simulink model "twozonevav"  (R2020a)
settings: Solver=FixedStepAuto  StartTime=0.0  StopTime=Inf  FixedStep=0.001  RelTol=1e-3
PostLoadFcn:
  | if any(exist('dsrtsu_mdlpostloadfcn', 'file') ~= 0), dsrtsu_mdlpostloadfcn('Execute', bdroot); end
InitFcn:
  | , if any(exist('rtifpga_mdlclblib', 'file') ~= 0), rtifpga_mdlclblib('Init', bdroot); end,
  | , if any(exist('dsmpb_private', 'file') ~= 0), dsmpb_private('dsmpb_mdlclblib', 'Init', bdroot); end,
libraries: dsmpblib x8
(part 2 of 3)

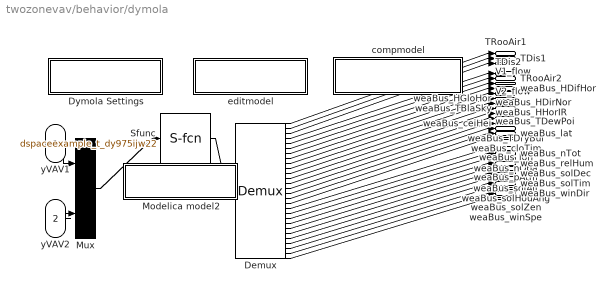
== system twozonevav/behavior/dymola ==
  yVAV1 : Inport
  yVAV2 : Inport  Port=2
  Demux : Demux  Outputs=[1;1;1;1;1;1;1;1;1;1;1;1;1;1;1;1;1;1;1;1;1;1;1;1;1;1;1;1]
  Dymola Settings : Subsystem  mask{ModelName=dSpaceExample.TwoZoneVAV, MoFileName=D:/github/dspace-modelica-example/dSpaceExample/TwoZoneVAV.mo, dSpace=, BusConnector=[], ResultFile=[], ResultFileOnline=[], ResultDt=[], Libs=:, bigobj=[], ImportFolder=[], guimode=[], ModelName2=[], forRuntime=[], MEXLoad=[], omitDescription=[], ResultName=dspaceexample_t_dy975ijw22}
      mask prompts: ModelName "Name of Dymola model"; MoFileName "File Name (including .mo)"; ResultFile "Create Result"; ResultFileOnline "Load result"; ResultDt "Result min dt"; Libs "Used Libraries"; bigobj "Compiler flag /bigobj"; ImportFolder "Import folder"; guimode "GUI mode flag"; ModelName2 "Model name for import mode"; forRuntime "Runtime export"; MEXLoad "Compiled S-function"; omitDescription "Omit description strings"; ResultName "Name of result file"
      mask Display: disp('Dymola Settings');
  Modelica model2 : Subsystem
      mask Display: disp('Change parameters');
  Mux : Mux  Inputs=[1;1]
  Sfunc : S-Function  Tag=975ijw22  FunctionName=dspaceexample_t_dy975ijw22  Parameters=[VRoo;zon1_S_;zon1_E_;zon1_W_;zon1_N_;zon1_matExtWal_absIR_a;zon1_matExtWal_absIR_b;zon1_matExtWal_absSol_a;zon1_matExtWal_absSol_b;zon1_matExtWal_roughness_10;zon1_matFlo_absIR_a;zon1_matFlo_absIR_b;zon1_matFlo_absSol_a;zon1_matFlo_absSol_b;zon1_matFlo_roughness_a;zon1_roof_absIR_a;zon1_roof_absIR_b;zon1_roof_absSol_a;zon1_roof_absSol_b;zon1_roof_roughness_a;zon1_window600_glass_1__x;zon1_window600_glass_1__k;zon1_window600_glass_1__t23;zon1_window600_glass_1__r24;zon1_window600_glass_1__r25;zon1_window600_glass_1__t26;zon1_window600_glass_1__a27;zon1_window600_glass_1__a28;zon1_window600_glass_2__x;zon1_window600_glass_2__k;zon1_window600_glass_2__t31;zon1_window600_glass_2__r32;zon1_window600_glass_2__r33;zon1_window600_glass_2__t34;zon1_window600_glass_2__a35;zon1_window600_glass_2__a36;zon1_window600_gas_1__x;zon1_window600_gas_1__a_k;zon1_window600_gas_1__b_k;zon1_window600_gas_1__a_m40;zon1_window600_gas_1__b_m41;zon1_window600_gas_1__a_c;zon1_window600_gas_1__b_c;zon1_window600_gas_1__MM;zon1_window600_gas_1__P0;zon1_window600_shade_tauS46;zon1_window600_shade_tauS47;zon1_window600_shade_rhoS48;zon1_window600_shade_rhoS49;zon1_window600_shade_absI50;zon1_window600_shade_absI51;zon1_window600_shade_tauI52;zon1_window600_shade_tauI53;zon1_window600_UFra;zon1_window600_absIRFra;zon1_window600_absSolFra;zon1_soi_A;zon1_soi_T_a_start;zon1_soi_T_b_start;zon1_roo_datConExt_1__bou60;zon1_roo_datConExt_1__A;zon1_roo_datConExt_2__bou62;zon1_roo_datConExt_2__A;zon1_roo_datConExt_3__bou64;zon1_roo_datConExt_3__A;zon1_roo_datConExt_4__bou66;zon1_roo_datConExt_4__A;zon1_roo_datConExtWin_1__68;zon1_roo_datConExtWin_1__69;zon1_roo_datConExtWin_1__70;zon1_roo_datConExtWin_1__71;zon1_roo_datConExtWin_1__72;zon1_roo_datConExtWin_1__73;zon1_roo_datConExtWin_1__74;zon1_roo_datConExtWin_1__75;zon1_roo_datConExtWin_1__76;zon1_roo_datConExtWin_1__77;zon1_roo_datConPar_1__azi;zon1_roo_datConPar_1__bou79;zon1_roo_datConPar_1__A;zon1_roo_datConBou_1__azi;zon1_roo_datConBou_1__bou82;zon1_roo_datConBou_1__A;zon1_roo_surBou_1__A;zon1_roo_surBou_1__absIR;zon1_roo_surBou_1__absSol;zon1_roo_surBou_1__bounda87;zon1_roo_dummyCon_absIR_a;zon1_roo_dummyCon_absIR_b;zon1_roo_dummyCon_absSol_90;zon1_roo_dummyCon_absSol_91;zon1_roo_dummyCon_roughne92;zon1_roo_dummyGlaSys_glas93;zon1_roo_dummyGlaSys_glas94;zon1_roo_dummyGlaSys_glas95;zon1_roo_dummyGlaSys_glas96;zon1_roo_dummyGlaSys_glas97;zon1_roo_dummyGlaSys_glas98;zon1_roo_dummyGlaSys_glas99;zon1_roo_dummyGlaSys_glas100;zon1_roo_dummyGlaSys_gas_101;zon1_roo_dummyGlaSys_gas_102;zon1_roo_dummyGlaSys_gas_103;zon1_roo_dummyGlaSys_gas_104;zon1_roo_dummyGlaSys_gas_105;zon1_roo_dummyGlaSys_gas_106;zon1_roo_dummyGlaSys_gas_107;zon1_roo_dummyGlaSys_gas_108;zon1_roo_dummyGlaSys_gas_109;zon1_roo_dummyGlaSys_shad110;zon1_roo_dummyGlaSys_shad111;zon1_roo_dummyGlaSys_shad112;zon1_roo_dummyGlaSys_shad113;zon1_roo_dummyGlaSys_shad114;zon1_roo_dummyGlaSys_shad115;zon1_roo_dummyGlaSys_shad116;zon1_roo_dummyGlaSys_shad117;zon1_roo_dummyGlaSys_UFra;zon1_roo_dummyGlaSys_absI119;zon1_roo_dummyGlaSys_absS120;zon1_roo_AFlo;zon1_roo_hRoo;zon1_roo_conExtWin_1__gla123;zon1_roo_conExtWin_1__win124;zon1_roo_conExtWin_1__win125;zon1_roo_conExtWin_1__win126;zon1_roo_conExtWin_1__win127;zon1_roo_hIntFixed;zon1_roo_hExtFixed;zon1_roo_bouConExt_HDifTi130;zon1_roo_bouConExt_HDifTi131;zon1_roo_bouConExt_HDifTi132;zon1_roo_bouConExt_HDifTi133;zon1_roo_bouConExt_HDifTi134;zon1_roo_bouConExt_HDifTi135;zon1_roo_bouConExt_HDifTi136;zon1_roo_bouConExt_HDifTi137;zon1_roo_bouConExt_HDifTi138;zon1_roo_bouConExt_HDifTi139;zon1_roo_bouConExt_HDifTi140;zon1_roo_bouConExt_HDifTi141;zon1_roo_bouConExtWin_con142;zon1_roo_bouConExtWin_con143;zon1_roo_bouConExtWin_HDi144;zon1_roo_bouConExtWin_HDi145;zon1_roo_bouConExtWin_HDi146;zon1_roo_bouConExtWin_con147;zon1_roo_air_datConExtWin148;zon1_roo_air_datConExtWin149;zon1_roo_air_dummyCon_abs150;zon1_roo_air_dummyCon_abs151;zon1_roo_air_dummyCon_abs152;zon1_roo_air_dummyCon_abs153;zon1_roo_air_dummyCon_rou154;zon1_roo_air_dummyGlaSys_155;zon1_roo_air_dummyGlaSys_156;zon1_roo_air_dummyGlaSys_157;zon1_roo_air_dummyGlaSys_158;zon1_roo_air_dummyGlaSys_159;zon1_roo_air_dummyGlaSys_160;zon1_roo_air_dummyGlaSys_161;zon1_roo_air_dummyGlaSys_162;zon1_roo_air_dummyGlaSys_163;zon1_roo_air_dummyGlaSys_164;zon1_roo_air_dummyGlaSys_165;zon1_roo_air_dummyGlaSys_166;zon1_roo_air_dummyGlaSys_167;zon1_roo_air_dummyGlaSys_168;zon1_roo_air_dummyGlaSys_169;zon1_roo_air_dummyGlaSys_170;zon1_roo_air_dummyGlaSys_171;zon1_roo_air_dummyGlaSys_172;zon1_roo_air_dummyGlaSys_173;zon1_roo_air_dummyGlaSys_174;zon1_roo_air_dummyGlaSys_175;zon1_roo_air_dummyGlaSys_176;zon1_roo_air_dummyGlaSys_177;zon1_roo_air_dummyGlaSys_178;zon1_roo_air_dummyGlaSys_179;zon1_roo_air_dummyGlaSys_180;zon1_roo_air_dummyGlaSys_181;zon1_roo_air_dummyGlaSys_182;zon1_roo_solRadExc_datCon183;zon1_roo_solRadExc_datCon184;zon1_roo_solRadExc_dummyC185;zon1_roo_solRadExc_dummyC186;zon1_roo_solRadExc_dummyC187;zon1_roo_solRadExc_dummyC188;zon1_roo_solRadExc_dummyC189;zon1_roo_solRadExc_dummyG190;zon1_roo_solRadExc_dummyG191;zon1_roo_solRadExc_dummyG192;zon1_roo_solRadExc_dummyG193;zon1_roo_solRadExc_dummyG194;zon1_roo_solRadExc_dummyG195;zon1_roo_solRadExc_dummyG196;zon1_roo_solRadExc_dummyG197;zon1_roo_solRadExc_dummyG198;zon1_roo_solRadExc_dummyG199;zon1_roo_solRadExc_dummyG200;zon1_roo_solRadExc_dummyG201;zon1_roo_solRadExc_dummyG202;zon1_roo_solRadExc_dummyG203;zon1_roo_solRadExc_dummyG204;zon1_roo_solRadExc_dummyG205;zon1_roo_solRadExc_dummyG206;zon1_roo_solRadExc_dummyG207;zon1_roo_solRadExc_dummyG208;zon1_roo_solRadExc_dummyG209;zon1_roo_solRadExc_dummyG210;zon1_roo_solRadExc_dummyG211;zon1_roo_solRadExc_dummyG212;zon1_roo_solRadExc_dummyG213;zon1_roo_solRadExc_dummyG214;zon1_roo_solRadExc_dummyG215;zon1_roo_solRadExc_dummyG216;zon1_roo_solRadExc_dummyG217;zon1_roo_irRadGai_datConE218;zon1_roo_irRadGai_datConE219;zon1_roo_irRadGai_dummyCo220;zon1_roo_irRadGai_dummyCo221;zon1_roo_irRadGai_dummyCo222;zon1_roo_irRadGai_dummyCo223;zon1_roo_irRadGai_dummyCo224;zon1_roo_irRadGai_dummyGl225;zon1_roo_irRadGai_dummyGl226;zon1_roo_irRadGai_dummyGl227;zon1_roo_irRadGai_dummyGl228;zon1_roo_irRadGai_dummyGl229;zon1_roo_irRadGai_dummyGl230;zon1_roo_irRadGai_dummyGl231;zon1_roo_irRadGai_dummyGl232;zon1_roo_irRadGai_dummyGl233;zon1_roo_irRadGai_dummyGl234;zon1_roo_irRadGai_dummyGl235;zon1_roo_irRadGai_dummyGl236;zon1_roo_irRadGai_dummyGl237;zon1_roo_irRadGai_dummyGl238;zon1_roo_irRadGai_dummyGl239;zon1_roo_irRadGai_dummyGl240;zon1_roo_irRadGai_dummyGl241;zon1_roo_irRadGai_dummyGl242;zon1_roo_irRadGai_dummyGl243;zon1_roo_irRadGai_dummyGl244;zon1_roo_irRadGai_dummyGl245;zon1_roo_irRadGai_dummyGl246;zon1_roo_irRadGai_dummyGl247;zon1_roo_irRadGai_dummyGl248;zon1_roo_irRadGai_dummyGl249;zon1_roo_irRadGai_dummyGl250;zon1_roo_irRadGai_dummyGl251;zon1_roo_irRadGai_dummyGl252;zon1_roo_irRadExc_datConE253;zon1_roo_irRadExc_datConE254;zon1_roo_irRadExc_dummyCo255;zon1_roo_irRadExc_dummyCo256;zon1_roo_irRadExc_dummyCo257;zon1_roo_irRadExc_dummyCo258;zon1_roo_irRadExc_dummyCo259;zon1_roo_irRadExc_dummyGl260;zon1_roo_irRadExc_dummyGl261;zon1_roo_irRadExc_dummyGl262;zon1_roo_irRadExc_dummyGl263;zon1_roo_irRadExc_dummyGl264;zon1_roo_irRadExc_dummyGl265;zon1_roo_irRadExc_dummyGl266;zon1_roo_irRadExc_dummyGl267;zon1_roo_irRadExc_dummyGl268;zon1_roo_irRadExc_dummyGl269;zon1_roo_irRadExc_dummyGl270;zon1_roo_irRadExc_dummyGl271;zon1_roo_irRadExc_dummyGl272;zon1_roo_irRadExc_dummyGl273;zon1_roo_irRadExc_dummyGl274;zon1_roo_irRadExc_dummyGl275;zon1_roo_irRadExc_dummyGl276;zon1_roo_irRadExc_dummyGl277;zon1_roo_irRadExc_dummyGl278;zon1_roo_irRadExc_dummyGl279;zon1_roo_irRadExc_dummyGl280;zon1_roo_irRadExc_dummyGl281;zon1_roo_irRadExc_dummyGl282;zon1_roo_irRadExc_dummyGl283;zon1_roo_irRadExc_dummyGl284;zon1_roo_irRadExc_dummyGl285;zon1_roo_irRadExc_dummyGl286;zon1_roo_irRadExc_dummyGl287;zon1_roo_irRadExc_T0;zon1_roo_radTem_datConExt289;zon1_roo_radTem_datConExt290;zon1_roo_radTem_dummyCon_291;zon1_roo_radTem_dummyCon_292;zon1_roo_radTem_dummyCon_293;zon1_roo_radTem_dummyCon_294;zon1_roo_radTem_dummyCon_295;zon1_roo_radTem_dummyGlaS296;zon1_roo_radTem_dummyGlaS297;zon1_roo_radTem_dummyGlaS298;zon1_roo_radTem_dummyGlaS299;zon1_roo_radTem_dummyGlaS300;zon1_roo_radTem_dummyGlaS301;zon1_roo_radTem_dummyGlaS302;zon1_roo_radTem_dummyGlaS303;zon1_roo_radTem_dummyGlaS304;zon1_roo_radTem_dummyGlaS305;zon1_roo_radTem_dummyGlaS306;zon1_roo_radTem_dummyGlaS307;zon1_roo_radTem_dummyGlaS308;zon1_roo_radTem_dummyGlaS309;zon1_roo_radTem_dummyGlaS310;zon1_roo_radTem_dummyGlaS311;zon1_roo_radTem_dummyGlaS312;zon1_roo_radTem_dummyGlaS313;zon1_roo_radTem_dummyGlaS314;zon1_roo_radTem_dummyGlaS315;zon1_roo_radTem_dummyGlaS316;zon1_roo_radTem_dummyGlaS317;zon1_roo_radTem_dummyGlaS318;zon1_roo_radTem_dummyGlaS319;zon1_roo_radTem_dummyGlaS320;zon1_roo_radTem_dummyGlaS321;zon1_roo_radTem_dummyGlaS322;zon1_roo_radTem_dummyGlaS323;zon1_roo_add_k1;zon1_roo_add_k2;zon1_roo_sumJFroWin_1__k;zon1_roo_p_start;zon1_roo_T_start;zon1_roo_X_start;zon1_qConGai_flow_k;zon1_qRadGai_flow_k;zon1_qLatGai_flow_k;zon1_TSoi_1__T;zon1_sinInf_m_flow;zon1_sinInf_x_pTphi_p;zon1_InfiltrationRate_k;zon1_souInf_m_flow;zon1_souInf_x_pTphi_p;zon1_intLoad_table;zon1_intLoad_verboseRead;zon1_intLoad_columns;zon1_intLoad_offset;zon1_intLoad_startTime;zon1_intLoad_timeEvents;coiSou_X;coiSou_T;res_sta_default_p;res_sta_default_T;res_sta_default_X;weaDat_lon;weaDat_lat;weaDat_wea_table;weaDat_wea_verboseRead;weaDat_wea_offset;weaDat_wea_startTime;weaDat_wea_timeEvents;sin_X;sin_p;sin_T;vav1_vav_sta_default_p;vav1_vav_sta_default_T;vav1_vav_sta_default_X;vav1_vav_riseTime;vav1_vav_y_start;vav1_vav_filter_gain;vav1_vav_filter_A_ripple;vav1_vav_filter_f_min;vav1_vav_filter_normalize368;vav1_vav_filter_x_start;vav1_vav_filter_u_nominal;vav1_vav_use_deltaM;vav1_vav_deltaM;vav1_vav_roundDuct;vav1_vav_ReC;vav1_vav_a;vav1_vav_b;vav1_vav_yL;vav1_vav_yU;vav1_vav_k1;vav1_vav_l;vav1_vav_l2;vav1_vav_deltax;vav1_vav_y_min;vav1_terHea_bal1_preDro_s384;vav1_terHea_bal1_preDro_s385;vav1_terHea_bal1_preDro_s386;vav1_terHea_bal2_preDro_s387;vav1_terHea_bal2_preDro_s388;vav1_terHea_delta;vav1_terHea_T_a1_nominal;vav1_terHea_T_a2_nominal;vav1_terHea_r_nominal;vav1_terHea_hA_n_w;vav1_terHea_hA_n_a;vav1_terHea_hA_T0_w;vav1_terHea_hA_T0_a;vav1_sinTer_X;vav1_sinTer_p;vav1_sinTer_T;vav1_souTer_X;vav1_souTer_m_flow;vav1_souTer_T;VSup1_T_start;VSup1_p_start;VSup1_X_start;TDisVAV1_T_start;TDisVAV1_TAmb;TDisVAV1_tauHeaTra;zer_k;vav2_vav_sta_default_p;vav2_vav_sta_default_T;vav2_vav_sta_default_X;vav2_vav_riseTime;vav2_vav_y_start;vav2_vav_filter_gain;vav2_vav_filter_A_ripple;vav2_vav_filter_f_min;vav2_vav_filter_normalize418;vav2_vav_filter_x_start;vav2_vav_filter_u_nominal;vav2_vav_use_deltaM;vav2_vav_deltaM;vav2_vav_roundDuct;vav2_vav_ReC;vav2_vav_a;vav2_vav_b;vav2_vav_yL;vav2_vav_yU;vav2_vav_k1;vav2_vav_l;vav2_vav_l2;vav2_vav_deltax;vav2_vav_y_min;vav2_terHea_bal1_preDro_s434;vav2_terHea_bal1_preDro_s435;vav2_terHea_bal1_preDro_s436;vav2_terHea_bal2_preDro_s437;vav2_terHea_bal2_preDro_s438;vav2_terHea_delta;vav2_terHea_T_a1_nominal;vav2_terHea_T_a2_nominal;vav2_terHea_r_nominal;vav2_terHea_hA_n_w;vav2_terHea_hA_n_a;vav2_terHea_hA_T0_w;vav2_terHea_hA_T0_a;vav2_sinTer_X;vav2_sinTer_p;vav2_sinTer_T;vav2_souTer_X;vav2_souTer_m_flow;vav2_souTer_T;TDisVAV2_T_start;TDisVAV2_TAmb;TDisVAV2_tauHeaTra;VSup2_T_start;VSup2_p_start;VSup2_X_start;zon2_S_;zon2_E_;zon2_W_;zon2_N_;zon2_matExtWal_absIR_a;zon2_matExtWal_absIR_b;zon2_matExtWal_absSol_a;zon2_matExtWal_absSol_b;zon2_matExtWal_roughness_467;zon2_matFlo_absIR_a;zon2_matFlo_absIR_b;zon2_matFlo_absSol_a;zon2_matFlo_absSol_b;zon2_matFlo_roughness_a;zon2_roof_absIR_a;zon2_roof_absIR_b;zon2_roof_absSol_a;zon2_roof_absSol_b;zon2_roof_roughness_a;zon2_window600_glass_1__x;zon2_window600_glass_1__k;zon2_window600_glass_1__t480;zon2_window600_glass_1__r481;zon2_window600_glass_1__r482;zon2_window600_glass_1__t483;zon2_window600_glass_1__a484;zon2_window600_glass_1__a485;zon2_window600_glass_2__x;zon2_window600_glass_2__k;zon2_window600_glass_2__t488;zon2_window600_glass_2__r489;zon2_window600_glass_2__r490;zon2_window600_glass_2__t491;zon2_window600_glass_2__a492;zon2_window600_glass_2__a493;zon2_window600_gas_1__x;zon2_window600_gas_1__a_k;zon2_window600_gas_1__b_k;zon2_window600_gas_1__a_m497;zon2_window600_gas_1__b_m498;zon2_window600_gas_1__a_c;zon2_window600_gas_1__b_c;zon2_window600_gas_1__MM;zon2_window600_gas_1__P0;zon2_window600_shade_tauS503;zon2_window600_shade_tauS504;zon2_window600_shade_rhoS505;zon2_window600_shade_rhoS506;zon2_window600_shade_absI507;zon2_window600_shade_absI508;zon2_window600_shade_tauI509;zon2_window600_shade_tauI510;zon2_window600_UFra;zon2_window600_absIRFra;zon2_window600_absSolFra;zon2_soi_A;zon2_soi_T_a_start;zon2_soi_T_b_start;zon2_roo_datConExt_1__bou517;zon2_roo_datConExt_1__A;zon2_roo_datConExt_2__bou519;zon2_roo_datConExt_2__A;zon2_roo_datConExt_3__bou521;zon2_roo_datConExt_3__A;zon2_roo_datConExt_4__bou523;zon2_roo_datConExt_4__A;zon2_roo_datConExtWin_1__525;zon2_roo_datConExtWin_1__526;zon2_roo_datConExtWin_1__527;zon2_roo_datConExtWin_1__528;zon2_roo_datConExtWin_1__529;zon2_roo_datConExtWin_1__530;zon2_roo_datConExtWin_1__531;zon2_roo_datConExtWin_1__532;zon2_roo_datConExtWin_1__533;zon2_roo_datConExtWin_1__534;zon2_roo_datConPar_1__azi;zon2_roo_datConPar_1__bou536;zon2_roo_datConPar_1__A;zon2_roo_datConBou_1__azi;zon2_roo_datConBou_1__bou539;zon2_roo_datConBou_1__A;zon2_roo_surBou_1__A;zon2_roo_surBou_1__absIR;zon2_roo_surBou_1__absSol;zon2_roo_surBou_1__bounda544;zon2_roo_dummyCon_absIR_a;zon2_roo_dummyCon_absIR_b;zon2_roo_dummyCon_absSol_547;zon2_roo_dummyCon_absSol_548;zon2_roo_dummyCon_roughne549;zon2_roo_dummyGlaSys_glas550;zon2_roo_dummyGlaSys_glas551;zon2_roo_dummyGlaSys_glas552;zon2_roo_dummyGlaSys_glas553;zon2_roo_dummyGlaSys_glas554;zon2_roo_dummyGlaSys_glas555;zon2_roo_dummyGlaSys_glas556;zon2_roo_dummyGlaSys_glas557;zon2_roo_dummyGlaSys_gas_558;zon2_roo_dummyGlaSys_gas_559;zon2_roo_dummyGlaSys_gas_560;zon2_roo_dummyGlaSys_gas_561;zon2_roo_dummyGlaSys_gas_562;zon2_roo_dummyGlaSys_gas_563;zon2_roo_dummyGlaSys_gas_564;zon2_roo_dummyGlaSys_gas_565;zon2_roo_dummyGlaSys_gas_566;zon2_roo_dummyGlaSys_shad567;zon2_roo_dummyGlaSys_shad568;zon2_roo_dummyGlaSys_shad569;zon2_roo_dummyGlaSys_shad570;zon2_roo_dummyGlaSys_shad571;zon2_roo_dummyGlaSys_shad572;zon2_roo_dummyGlaSys_shad573;zon2_roo_dummyGlaSys_shad574;zon2_roo_dummyGlaSys_UFra;zon2_roo_dummyGlaSys_absI576;zon2_roo_dummyGlaSys_absS577;zon2_roo_AFlo;zon2_roo_hRoo;zon2_roo_conExtWin_1__gla580;zon2_roo_conExtWin_1__win581;zon2_roo_conExtWin_1__win582;zon2_roo_conExtWin_1__win583;zon2_roo_conExtWin_1__win584;zon2_roo_hIntFixed;zon2_roo_hExtFixed;zon2_roo_bouConExt_HDifTi587;zon2_roo_bouConExt_HDifTi588;zon2_roo_bouConExt_HDifTi589;zon2_roo_bouConExt_HDifTi590;zon2_roo_bouConExt_HDifTi591;zon2_roo_bouConExt_HDifTi592;zon2_roo_bouConExt_HDifTi593;zon2_roo_bouConExt_HDifTi594;zon2_roo_bouConExt_HDifTi595;zon2_roo_bouConExt_HDifTi596;zon2_roo_bouConExt_HDifTi597;zon2_roo_bouConExt_HDifTi598;zon2_roo_bouConExtWin_con599;zon2_roo_bouConExtWin_con600;zon2_roo_bouConExtWin_HDi601;zon2_roo_bouConExtWin_HDi602;zon2_roo_bouConExtWin_HDi603;zon2_roo_bouConExtWin_con604;zon2_roo_air_datConExtWin605;zon2_roo_air_datConExtWin606;zon2_roo_air_dummyCon_abs607;zon2_roo_air_dummyCon_abs608;zon2_roo_air_dummyCon_abs609;zon2_roo_air_dummyCon_abs610;zon2_roo_air_dummyCon_rou611;zon2_roo_air_dummyGlaSys_612;zon2_roo_air_dummyGlaSys_613;zon2_roo_air_dummyGlaSys_614;zon2_roo_air_dummyGlaSys_615;zon2_roo_air_dummyGlaSys_616;zon2_roo_air_dummyGlaSys_617;zon2_roo_air_dummyGlaSys_618;zon2_roo_air_dummyGlaSys_619;zon2_roo_air_dummyGlaSys_620;zon2_roo_air_dummyGlaSys_621;zon2_roo_air_dummyGlaSys_622;zon2_roo_air_dummyGlaSys_623;zon2_roo_air_dummyGlaSys_624;zon2_roo_air_dummyGlaSys_625;zon2_roo_air_dummyGlaSys_626;zon2_roo_air_dummyGlaSys_627;zon2_roo_air_dummyGlaSys_628;zon2_roo_air_dummyGlaSys_629;zon2_roo_air_dummyGlaSys_630;zon2_roo_air_dummyGlaSys_631;zon2_roo_air_dummyGlaSys_632;zon2_roo_air_dummyGlaSys_633;zon2_roo_air_dummyGlaSys_634;zon2_roo_air_dummyGlaSys_635;zon2_roo_air_dummyGlaSys_636;zon2_roo_air_dummyGlaSys_637;zon2_roo_air_dummyGlaSys_638;zon2_roo_air_dummyGlaSys_639;zon2_roo_solRadExc_datCon640;zon2_roo_solRadExc_datCon641;zon2_roo_solRadExc_dummyC642;zon2_roo_solRadExc_dummyC643;zon2_roo_solRadExc_dummyC644;zon2_roo_solRadExc_dummyC645;zon2_roo_solRadExc_dummyC646;zon2_roo_solRadExc_dummyG647;zon2_roo_solRadExc_dummyG648;zon2_roo_solRadExc_dummyG649;zon2_roo_solRadExc_dummyG650;zon2_roo_solRadExc_dummyG651;zon2_roo_solRadExc_dummyG652;zon2_roo_solRadExc_dummyG653;zon2_roo_solRadExc_dummyG654;zon2_roo_solRadExc_dummyG655;zon2_roo_solRadExc_dummyG656;zon2_roo_solRadExc_dummyG657;zon2_roo_solRadExc_dummyG658;zon2_roo_solRadExc_dummyG659;zon2_roo_solRadExc_dummyG660;zon2_roo_solRadExc_dummyG661;zon2_roo_solRadExc_dummyG662;zon2_roo_solRadExc_dummyG663;zon2_roo_solRadExc_dummyG664;zon2_roo_solRadExc_dummyG665;zon2_roo_solRadExc_dummyG666;zon2_roo_solRadExc_dummyG667;zon2_roo_solRadExc_dummyG668;zon2_roo_solRadExc_dummyG669;zon2_roo_solRadExc_dummyG670;zon2_roo_solRadExc_dummyG671;zon2_roo_solRadExc_dummyG672;zon2_roo_solRadExc_dummyG673;zon2_roo_solRadExc_dummyG674;zon2_roo_irRadGai_datConE675;zon2_roo_irRadGai_datConE676;zon2_roo_irRadGai_dummyCo677;zon2_roo_irRadGai_dummyCo678;zon2_roo_irRadGai_dummyCo679;zon2_roo_irRadGai_dummyCo680;zon2_roo_irRadGai_dummyCo681;zon2_roo_irRadGai_dummyGl682;zon2_roo_irRadGai_dummyGl683;zon2_roo_irRadGai_dummyGl684;zon2_roo_irRadGai_dummyGl685;zon2_roo_irRadGai_dummyGl686;zon2_roo_irRadGai_dummyGl687;zon2_roo_irRadGai_dummyGl688;zon2_roo_irRadGai_dummyGl689;zon2_roo_irRadGai_dummyGl690;zon2_roo_irRadGai_dummyGl691;zon2_roo_irRadGai_dummyGl692;zon2_roo_irRadGai_dummyGl693;zon2_roo_irRadGai_dummyGl694;zon2_roo_irRadGai_dummyGl695;zon2_roo_irRadGai_dummyGl696;zon2_roo_irRadGai_dummyGl697;zon2_roo_irRadGai_dummyGl698;zon2_roo_irRadGai_dummyGl699;zon2_roo_irRadGai_dummyGl700;zon2_roo_irRadGai_dummyGl701;zon2_roo_irRadGai_dummyGl702;zon2_roo_irRadGai_dummyGl703;zon2_roo_irRadGai_dummyGl704;zon2_roo_irRadGai_dummyGl705;zon2_roo_irRadGai_dummyGl706;zon2_roo_irRadGai_dummyGl707;zon2_roo_irRadGai_dummyGl708;zon2_roo_irRadGai_dummyGl709;zon2_roo_irRadExc_datConE710;zon2_roo_irRadExc_datConE711;zon2_roo_irRadExc_dummyCo712;zon2_roo_irRadExc_dummyCo713;zon2_roo_irRadExc_dummyCo714;zon2_roo_irRadExc_dummyCo715;zon2_roo_irRadExc_dummyCo716;zon2_roo_irRadExc_dummyGl717;zon2_roo_irRadExc_dummyGl718;zon2_roo_irRadExc_dummyGl719;zon2_roo_irRadExc_dummyGl720;zon2_roo_irRadExc_dummyGl721;zon2_roo_irRadExc_dummyGl722;zon2_roo_irRadExc_dummyGl723;zon2_roo_irRadExc_dummyGl724;zon2_roo_irRadExc_dummyGl725;zon2_roo_irRadExc_dummyGl726;zon2_roo_irRadExc_dummyGl727;zon2_roo_irRadExc_dummyGl728;zon2_roo_irRadExc_dummyGl729;zon2_roo_irRadExc_dummyGl730;zon2_roo_irRadExc_dummyGl731;zon2_roo_irRadExc_dummyGl732;zon2_roo_irRadExc_dummyGl733;zon2_roo_irRadExc_dummyGl734;zon2_roo_irRadExc_dummyGl735;zon2_roo_irRadExc_dummyGl736;zon2_roo_irRadExc_dummyGl737;zon2_roo_irRadExc_dummyGl738;zon2_roo_irRadExc_dummyGl739;zon2_roo_irRadExc_dummyGl740;zon2_roo_irRadExc_dummyGl741;zon2_roo_irRadExc_dummyGl742;zon2_roo_irRadExc_dummyGl743;zon2_roo_irRadExc_dummyGl744;zon2_roo_irRadExc_T0;zon2_roo_radTem_datConExt746;zon2_roo_radTem_datConExt747;zon2_roo_radTem_dummyCon_748;zon2_roo_radTem_dummyCon_749;zon2_roo_radTem_dummyCon_750;zon2_roo_radTem_dummyCon_751;zon2_roo_radTem_dummyCon_752;zon2_roo_radTem_dummyGlaS753;zon2_roo_radTem_dummyGlaS754;zon2_roo_radTem_dummyGlaS755;zon2_roo_radTem_dummyGlaS756;zon2_roo_radTem_dummyGlaS757;zon2_roo_radTem_dummyGlaS758;zon2_roo_radTem_dummyGlaS759;zon2_roo_radTem_dummyGlaS760;zon2_roo_radTem_dummyGlaS761;zon2_roo_radTem_dummyGlaS762;zon2_roo_radTem_dummyGlaS763;zon2_roo_radTem_dummyGlaS764;zon2_roo_radTem_dummyGlaS765;zon2_roo_radTem_dummyGlaS766;zon2_roo_radTem_dummyGlaS767;zon2_roo_radTem_dummyGlaS768;zon2_roo_radTem_dummyGlaS769;zon2_roo_radTem_dummyGlaS770;zon2_roo_radTem_dummyGlaS771;zon2_roo_radTem_dummyGlaS772;zon2_roo_radTem_dummyGlaS773;zon2_roo_radTem_dummyGlaS774;zon2_roo_radTem_dummyGlaS775;zon2_roo_radTem_dummyGlaS776;zon2_roo_radTem_dummyGlaS777;zon2_roo_radTem_dummyGlaS778;zon2_roo_radTem_dummyGlaS779;zon2_roo_radTem_dummyGlaS780;zon2_roo_add_k1;zon2_roo_add_k2;zon2_roo_sumJFroWin_1__k;zon2_roo_p_start;zon2_roo_T_start;zon2_roo_X_start;zon2_qConGai_flow_k;zon2_qRadGai_flow_k;zon2_qLatGai_flow_k;zon2_TSoi_1__T;zon2_sinInf_m_flow;zon2_sinInf_x_pTphi_p;zon2_InfiltrationRate_k;zon2_souInf_m_flow;zon2_souInf_x_pTphi_p;zon2_intLoad_table;zon2_intLoad_verboseRead;zon2_intLoad_columns;zon2_intLoad_offset;zon2_intLoad_startTime;zon2_intLoad_timeEvents;zon1_roo_conExtWin_1__win802;zon1_roo_conExtWin_1__win803;zon1_roo_conExtWin_1__win804;zon2_roo_conExtWin_1__win805;zon2_roo_conExtWin_1__win806;zon2_roo_conExtWin_1__win807],[]  PortCounts=[1;1]  SFunctionDeploymentMode=off  EnableBusSupport=off  mask{VRoo=129.6, zon1_S_=0, zon1_E_=-1.5707963267949, zon1_W_=1.5707963267949, zon1_N_=3.14159265358979, zon1_matExtWal_absIR_a=0.9, zon1_matExtWal_absIR_b=0.9, zon1_matExtWal_absSol_a=0.6, zon1_matExtWal_absSol_b=0.6, zon1_matExtWal_roughness_10=3, zon1_matFlo_absIR_a=0.9, zon1_matFlo_absIR_b=0.9, zon1_matFlo_absSol_a=0.6, zon1_matFlo_absSol_b=0.6, zon1_matFlo_roughness_a=3, zon1_roof_absIR_a=0.9, zon1_roof_absIR_b=0.9, zon1_roof_absSol_a=0.6, zon1_roof_absSol_b=0.6, zon1_roof_roughness_a=3, zon1_window600_glass_1__x=0.003175, zon1_window600_glass_1__k=1.06, zon1_window600_glass_1__t23=0.86156, zon1_window600_glass_1__r24=0.0434, zon1_window600_glass_1__r25=0.0434, zon1_window600_glass_1__t26=0, zon1_window600_glass_1__a27=0.9, zon1_window600_glass_1__a28=0.9, zon1_window600_glass_2__x=0.003175, zon1_window600_glass_2__k=1.06, zon1_window600_glass_2__t31=0.86156, zon1_window600_glass_2__r32=0.0434, zon1_window600_glass_2__r33=0.0434, zon1_window600_glass_2__t34=0, zon1_window600_glass_2__a35=0.9, zon1_window600_glass_2__a36=0.9, zon1_window600_gas_1__x=0.013, zon1_window600_gas_1__a_k=0.002873, zon1_window600_gas_1__b_k=7.76e-05, zon1_window600_gas_1__a_m40=3.723e-06, zon1_window600_gas_1__b_m41=4.94e-08, zon1_window600_gas_1__a_c=1002.737, zon1_window600_gas_1__b_c=0.012324, zon1_window600_gas_1__MM=0.02897, zon1_window600_gas_1__P0=101325, zon1_window600_shade_tauS46=0.1, zon1_window600_shade_tauS47=0.1, zon1_window600_shade_rhoS48=0.8, zon1_window600_shade_rhoS49=0.8, zon1_window600_shade_absI50=0.84, zon1_window600_shade_absI51=0.84, zon1_window600_shade_tauI52=0, zon1_window600_shade_tauI53=0, zon1_window600_UFra=3, zon1_window600_absIRFra=0.8, zon1_window600_absSolFra=0.5, zon1_soi_A=48, zon1_soi_T_a_start=283.15, zon1_soi_T_b_start=283.75, zon1_roo_datConExt_1__bou60=1, zon1_roo_datConExt_1__A=48, zon1_roo_datConExt_2__bou62=1, zon1_roo_datConExt_2__A=16.2, zon1_roo_datConExt_3__bou64=1, zon1_roo_datConExt_3__A=16.2, zon1_roo_datConExt_4__bou66=1, zon1_roo_datConExt_4__A=21.6, zon1_roo_datConExtWin_1__68=1, zon1_roo_datConExtWin_1__69=21.6, zon1_roo_datConExtWin_1__70=2, zon1_roo_datConExtWin_1__71=6, zon1_roo_datConExtWin_1__72=0.001, zon1_roo_datConExtWin_1__73=0, zon1_roo_datConExtWin_1__74=0, zon1_roo_datConExtWin_1__75=0, zon1_roo_datConExtWin_1__76=0, zon1_roo_datConExtWin_1__77=0, zon1_roo_datConPar_1__azi=0, zon1_roo_datConPar_1__bou79=1, zon1_roo_datConPar_1__A=0, zon1_roo_datConBou_1__azi=0, zon1_roo_datConBou_1__bou82=1, zon1_roo_datConBou_1__A=48, zon1_roo_surBou_1__A=0, zon1_roo_surBou_1__absIR=0.84, zon1_roo_surBou_1__absSol=0.84, zon1_roo_surBou_1__bounda87=1, zon1_roo_dummyCon_absIR_a=0.9, zon1_roo_dummyCon_absIR_b=0.9, zon1_roo_dummyCon_absSol_90=0.5, zon1_roo_dummyCon_absSol_91=0.5, zon1_roo_dummyCon_roughne92=3, zon1_roo_dummyGlaSys_glas93=0.003, zon1_roo_dummyGlaSys_glas94=1, zon1_roo_dummyGlaSys_glas95=0.834, zon1_roo_dummyGlaSys_glas96=0.075, zon1_roo_dummyGlaSys_glas97=0.075, zon1_roo_dummyGlaSys_glas98=0, zon1_roo_dummyGlaSys_glas99=0.84, zon1_roo_dummyGlaSys_glas100=0.84, zon1_roo_dummyGlaSys_gas_101=-1, zon1_roo_dummyGlaSys_gas_102=0.002873, zon1_roo_dummyGlaSys_gas_103=7.76e-05, zon1_roo_dummyGlaSys_gas_104=3.723e-06, zon1_roo_dummyGlaSys_gas_105=4.94e-08, zon1_roo_dummyGlaSys_gas_106=1002.737, zon1_roo_dummyGlaSys_gas_107=0.012324, zon1_roo_dummyGlaSys_gas_108=0.02897, zon1_roo_dummyGlaSys_gas_109=101325, zon1_roo_dummyGlaSys_shad110=0.1, zon1_roo_dummyGlaSys_shad111=0.1, zon1_roo_dummyGlaSys_shad112=0.8, zon1_roo_dummyGlaSys_shad113=0.8, zon1_roo_dummyGlaSys_shad114=0.84, zon1_roo_dummyGlaSys_shad115=0.84, zon1_roo_dummyGlaSys_shad116=0, zon1_roo_dummyGlaSys_shad117=0, zon1_roo_dummyGlaSys_UFra=3, zon1_roo_dummyGlaSys_absI119=0.8, zon1_roo_dummyGlaSys_absS120=0.5, zon1_roo_AFlo=48, zon1_roo_hRoo=2.7, zon1_roo_conExtWin_1__gla123=0, zon1_roo_conExtWin_1__win124=1, zon1_roo_conExtWin_1__win125=3, zon1_roo_conExtWin_1__win126=331.4, zon1_roo_conExtWin_1__win127=1, zon1_roo_hIntFixed=3, zon1_roo_hExtFixed=10, zon1_roo_bouConExt_HDifTi130=0.2, zon1_roo_bouConExt_HDifTi131=1, zon1_roo_bouConExt_HDifTi132=1, zon1_roo_bouConExt_HDifTi133=0.2, zon1_roo_bouConExt_HDifTi134=1, zon1_roo_bouConExt_HDifTi135=1, zon1_roo_bouConExt_HDifTi136=0.2, zon1_roo_bouConExt_HDifTi137=1, zon1_roo_bouConExt_HDifTi138=1, zon1_roo_bouConExt_HDifTi139=0.2, zon1_roo_bouConExt_HDifTi140=1, zon1_roo_bouConExt_HDifTi141=1, zon1_roo_bouConExtWin_con142=0, zon1_roo_bouConExtWin_con143=0, zon1_roo_bouConExtWin_HDi144=0.2, zon1_roo_bouConExtWin_HDi145=1, zon1_roo_bouConExtWin_HDi146=1, zon1_roo_bouConExtWin_con147=293.15, zon1_roo_air_datConExtWin148=0, zon1_roo_air_datConExtWin149=0, zon1_roo_air_dummyCon_abs150=0.9, zon1_roo_air_dummyCon_abs151=0.9, zon1_roo_air_dummyCon_abs152=0.5, zon1_roo_air_dummyCon_abs153=0.5, zon1_roo_air_dummyCon_rou154=3, zon1_roo_air_dummyGlaSys_155=0.003, zon1_roo_air_dummyGlaSys_156=1, zon1_roo_air_dummyGlaSys_157=0.834, zon1_roo_air_dummyGlaSys_158=0.075, zon1_roo_air_dummyGlaSys_159=0.075, zon1_roo_air_dummyGlaSys_160=0, zon1_roo_air_dummyGlaSys_161=0.84, zon1_roo_air_dummyGlaSys_162=0.84, zon1_roo_air_dummyGlaSys_163=-1, zon1_roo_air_dummyGlaSys_164=0.002873, zon1_roo_air_dummyGlaSys_165=7.76e-05, zon1_roo_air_dummyGlaSys_166=3.723e-06, zon1_roo_air_dummyGlaSys_167=4.94e-08, zon1_roo_air_dummyGlaSys_168=1002.737, zon1_roo_air_dummyGlaSys_169=0.012324, zon1_roo_air_dummyGlaSys_170=0.02897, zon1_roo_air_dummyGlaSys_171=101325, zon1_roo_air_dummyGlaSys_172=0.1, zon1_roo_air_dummyGlaSys_173=0.1, zon1_roo_air_dummyGlaSys_174=0.8, zon1_roo_air_dummyGlaSys_175=0.8, zon1_roo_air_dummyGlaSys_176=0.84, zon1_roo_air_dummyGlaSys_177=0.84, zon1_roo_air_dummyGlaSys_178=0, zon1_roo_air_dummyGlaSys_179=0, zon1_roo_air_dummyGlaSys_180=3, zon1_roo_air_dummyGlaSys_181=0.8, zon1_roo_air_dummyGlaSys_182=0.5, zon1_roo_solRadExc_datCon183=0, zon1_roo_solRadExc_datCon184=0, zon1_roo_solRadExc_dummyC185=0.9, zon1_roo_solRadExc_dummyC186=0.9, zon1_roo_solRadExc_dummyC187=0.5, zon1_roo_solRadExc_dummyC188=0.5, zon1_roo_solRadExc_dummyC189=3, zon1_roo_solRadExc_dummyG190=0.003, zon1_roo_solRadExc_dummyG191=1, zon1_roo_solRadExc_dummyG192=0.834, zon1_roo_solRadExc_dummyG193=0.075, zon1_roo_solRadExc_dummyG194=0.075, zon1_roo_solRadExc_dummyG195=0, zon1_roo_solRadExc_dummyG196=0.84, zon1_roo_solRadExc_dummyG197=0.84, zon1_roo_solRadExc_dummyG198=-1, zon1_roo_solRadExc_dummyG199=0.002873, zon1_roo_solRadExc_dummyG200=7.76e-05, zon1_roo_solRadExc_dummyG201=3.723e-06, zon1_roo_solRadExc_dummyG202=4.94e-08, zon1_roo_solRadExc_dummyG203=1002.737, zon1_roo_solRadExc_dummyG204=0.012324, zon1_roo_solRadExc_dummyG205=0.02897, zon1_roo_solRadExc_dummyG206=101325, zon1_roo_solRadExc_dummyG207=0.1, zon1_roo_solRadExc_dummyG208=0.1, zon1_roo_solRadExc_dummyG209=0.8, zon1_roo_solRadExc_dummyG210=0.8, zon1_roo_solRadExc_dummyG211=0.84, zon1_roo_solRadExc_dummyG212=0.84, zon1_roo_solRadExc_dummyG213=0, zon1_roo_solRadExc_dummyG214=0, zon1_roo_solRadExc_dummyG215=3, zon1_roo_solRadExc_dummyG216=0.8, zon1_roo_solRadExc_dummyG217=0.5, zon1_roo_irRadGai_datConE218=0, zon1_roo_irRadGai_datConE219=0, zon1_roo_irRadGai_dummyCo220=0.9, zon1_roo_irRadGai_dummyCo221=0.9, zon1_roo_irRadGai_dummyCo222=0.5, zon1_roo_irRadGai_dummyCo223=0.5, zon1_roo_irRadGai_dummyCo224=3, zon1_roo_irRadGai_dummyGl225=0.003, zon1_roo_irRadGai_dummyGl226=1, zon1_roo_irRadGai_dummyGl227=0.834, zon1_roo_irRadGai_dummyGl228=0.075, zon1_roo_irRadGai_dummyGl229=0.075, zon1_roo_irRadGai_dummyGl230=0, zon1_roo_irRadGai_dummyGl231=0.84, zon1_roo_irRadGai_dummyGl232=0.84, zon1_roo_irRadGai_dummyGl233=-1, zon1_roo_irRadGai_dummyGl234=0.002873, zon1_roo_irRadGai_dummyGl235=7.76e-05, zon1_roo_irRadGai_dummyGl236=3.723e-06, zon1_roo_irRadGai_dummyGl237=4.94e-08, zon1_roo_irRadGai_dummyGl238=1002.737, zon1_roo_irRadGai_dummyGl239=0.012324, zon1_roo_irRadGai_dummyGl240=0.02897, zon1_roo_irRadGai_dummyGl241=101325, zon1_roo_irRadGai_dummyGl242=0.1, zon1_roo_irRadGai_dummyGl243=0.1, zon1_roo_irRadGai_dummyGl244=0.8, zon1_roo_irRadGai_dummyGl245=0.8, zon1_roo_irRadGai_dummyGl246=0.84, zon1_roo_irRadGai_dummyGl247=0.84, zon1_roo_irRadGai_dummyGl248=0, zon1_roo_irRadGai_dummyGl249=0, zon1_roo_irRadGai_dummyGl250=3, zon1_roo_irRadGai_dummyGl251=0.8, zon1_roo_irRadGai_dummyGl252=0.5, zon1_roo_irRadExc_datConE253=0, zon1_roo_irRadExc_datConE254=0, zon1_roo_irRadExc_dummyCo255=0.9, zon1_roo_irRadExc_dummyCo256=0.9, zon1_roo_irRadExc_dummyCo257=0.5, zon1_roo_irRadExc_dummyCo258=0.5, zon1_roo_irRadExc_dummyCo259=3, zon1_roo_irRadExc_dummyGl260=0.003, zon1_roo_irRadExc_dummyGl261=1, zon1_roo_irRadExc_dummyGl262=0.834, zon1_roo_irRadExc_dummyGl263=0.075, zon1_roo_irRadExc_dummyGl264=0.075, zon1_roo_irRadExc_dummyGl265=0, zon1_roo_irRadExc_dummyGl266=0.84, zon1_roo_irRadExc_dummyGl267=0.84, zon1_roo_irRadExc_dummyGl268=-1, zon1_roo_irRadExc_dummyGl269=0.002873, zon1_roo_irRadExc_dummyGl270=7.76e-05, zon1_roo_irRadExc_dummyGl271=3.723e-06, zon1_roo_irRadExc_dummyGl272=4.94e-08, zon1_roo_irRadExc_dummyGl273=1002.737, zon1_roo_irRadExc_dummyGl274=0.012324, zon1_roo_irRadExc_dummyGl275=0.02897, zon1_roo_irRadExc_dummyGl276=101325, zon1_roo_irRadExc_dummyGl277=0.1, zon1_roo_irRadExc_dummyGl278=0.1, zon1_roo_irRadExc_dummyGl279=0.8, zon1_roo_irRadExc_dummyGl280=0.8, zon1_roo_irRadExc_dummyGl281=0.84, zon1_roo_irRadExc_dummyGl282=0.84, zon1_roo_irRadExc_dummyGl283=0, zon1_roo_irRadExc_dummyGl284=0, zon1_roo_irRadExc_dummyGl285=3, zon1_roo_irRadExc_dummyGl286=0.8, zon1_roo_irRadExc_dummyGl287=0.5, zon1_roo_irRadExc_T0=293.15, zon1_roo_radTem_datConExt289=0, zon1_roo_radTem_datConExt290=0, zon1_roo_radTem_dummyCon_291=0.9, zon1_roo_radTem_dummyCon_292=0.9, zon1_roo_radTem_dummyCon_293=0.5, zon1_roo_radTem_dummyCon_294=0.5, zon1_roo_radTem_dummyCon_295=3, zon1_roo_radTem_dummyGlaS296=0.003, zon1_roo_radTem_dummyGlaS297=1, zon1_roo_radTem_dummyGlaS298=0.834, zon1_roo_radTem_dummyGlaS299=0.075, zon1_roo_radTem_dummyGlaS300=0.075, zon1_roo_radTem_dummyGlaS301=0, zon1_roo_radTem_dummyGlaS302=0.84, zon1_roo_radTem_dummyGlaS303=0.84, zon1_roo_radTem_dummyGlaS304=-1, zon1_roo_radTem_dummyGlaS305=0.002873, zon1_roo_radTem_dummyGlaS306=7.76e-05, zon1_roo_radTem_dummyGlaS307=3.723e-06, zon1_roo_radTem_dummyGlaS308=4.94e-08, zon1_roo_radTem_dummyGlaS309=1002.737, zon1_roo_radTem_dummyGlaS310=0.012324, zon1_roo_radTem_dummyGlaS311=0.02897, zon1_roo_radTem_dummyGlaS312=101325, zon1_roo_radTem_dummyGlaS313=0.1, zon1_roo_radTem_dummyGlaS314=0.1, zon1_roo_radTem_dummyGlaS315=0.8, zon1_roo_radTem_dummyGlaS316=0.8, zon1_roo_radTem_dummyGlaS317=0.84, zon1_roo_radTem_dummyGlaS318=0.84, zon1_roo_radTem_dummyGlaS319=0, zon1_roo_radTem_dummyGlaS320=0, zon1_roo_radTem_dummyGlaS321=3, zon1_roo_radTem_dummyGlaS322=0.8, zon1_roo_radTem_dummyGlaS323=0.5, zon1_roo_add_k1=1, zon1_roo_add_k2=1, zon1_roo_sumJFroWin_1__k=1, zon1_roo_p_start=101325, zon1_roo_T_start=293.15, zon1_roo_X_start=[0.01; 0.99], zon1_qConGai_flow_k=4, zon1_qRadGai_flow_k=6, zon1_qLatGai_flow_k=2, zon1_TSoi_1__T=283.15, zon1_sinInf_m_flow=0, zon1_sinInf_x_pTphi_p=101325, zon1_InfiltrationRate_k=0.018, zon1_souInf_m_flow=0, zon1_souInf_x_pTphi_p=101325, zon1_intLoad_table=[0; 0.1; 28800; 0.1; 28800; 1; 64800; 1; 64800; 0.1; 86400; 0.1], zon1_intLoad_verboseRead=1, zon1_intLoad_columns=2, zon1_intLoad_offset=0, zon1_intLoad_startTime=0, zon1_intLoad_timeEvents=1, coiSou_X=[0.01; 0.99], coiSou_T=285.15, res_sta_default_p=101325, res_sta_default_T=293.15, res_sta_default_X=[0.01; 0.99], weaDat_lon=-1.534493, weaDat_lat=0.732689, weaDat_wea_table=[18316800; 166.213759539879; 354.348815343151; 463.524070844258; 406.70098500709; 290.921466566112; 292.375845295109; 299.777957864004; 294.719073987987; 1811.50684931507; 18316800; 0.463695339144093; 0.478209325712021; 0.643483357886745; 0.672020459828311; 0.315289432871832; 1328.90383200449; 18316939.6438356; 0.898775910677975; 2.39215084951218; 2.67854051394005; 0.732689201831818; -1.5344934463501; 101325; 18320400; 163.45642842332; 400.847059336971; 500.896302872053; 404.841077970043; 290.610253460331; 292.201656463484; 299.723268343433; 294.595035361373; 1829.77168949772; 18320400; 0.431941915524605; 0.445049508045253; 0.638649696764881; 0.705186722757609; 0.315101156019729; 1329.16564216788; 18320539.8721461; 0.865609647748677; 2.33288803329206; 2.63798426166517; 0.732689201831818; -1.5344934463501; 101325; 18324000; 160.699097306761; 447.345303330792; 538.268534899847; 402.981170932996; 290.29904035455; 292.027467631858; 299.668578822863; 294.470996734759; 1848.03652968037; 18324000; 0.400188491905117; 0.411889690378485; 0.633816035643016; 0.738352985686908; 0.314912879167626; 1329.42745233126; 18324140.1004566; 0.832443384819379; 2.27362521707195; 2.59742800939029; 0.732689201831818; -1.5344934463501; 101325; 18327600; 157.941766190202; 493.843547324612; 575.640766927641; 401.121263895949; 289.987827248769; 291.853278800233; 299.613889302293; 294.346958108144; 1866.30136986301; 18327600; 0.368435068285628; 0.378729872711717; 0.628982374521151; 0.771519248616205; 0.314724602315524; 1329.68926249465; 18327740.3287671; 0.799277121890081; 2.21436240085184; 2.5568717571154; 0.732689201831818; -1.5344934463501; 101325; 18331200; 155.184435073643; 540.341791318432; 613.012998955435; 399.261356858902; 289.676614142988; 291.679089968607; 299.559199781723; 294.22291948153; 1884.56621004566; 18331200; 0.33668164466614; 0.345570055044949; 0.624148713399286; 0.804685511545504; 0.314536325463421; 1329.95107265803; 18331340.5570776; 0.766110858960783; 2.15509958463172; 2.51631550484052; 0.732689201831818; -1.5344934463501; 101325; 18334800; 152.427103957085; 586.840035312252; 650.385230983229; 397.401449821855; 289.365401037208; 291.504901136982; 299.504510261152; 294.098880854916; 1902.83105022831; 18334800; 0.304928221046652; 0.312410237378181; 0.619315052277421; 0.837851774474802; 0.314348048611319; 1330.21288282142; 18334940.7853881; 0.732944596031485; 2.09583676841161; 2.47575925256564; 0.732689201831818; -1.5344934463501; 101325; 18338400; 149.669772840526; 633.338279306072; 687.757463011023; 395.541542784808; 289.054187931427; 291.330712305356; 299.449820740582; 293.974842228302; 1921.09589041096; 18338400; 0.273174797427164; 0.279250419711413; 0.614481391155556; 0.8710180374041; 0.314159771759216; 1330.4746929848; 18338541.0136986; 0.699778333102187; 2.0365739521915; 2.43520300029075; 0.732689201831818; -1.5344934463501; 101325; 18342000; 146.912441723967; 679.836523299892; 725.129695038817; 393.681635747762; 288.742974825646; 291.156523473731; 299.395131220012; 293.850803601687; 1939.36073059361; 18342000; 0.241421373807676; 0.246090602044646; 0.609647730033692; 0.904184300333398; 0.313971494907114; 1330.73650314819; 18342141.2420091; 0.666612070172889; 1.97731113597138; 2.39464674801587; 0.732689201831818; -1.5344934463501; 101325; 18345600; 144.155110607408; 726.334767293712; 762.501927066611; 391.821728710715; 288.431761719865; 290.982334642105; 299.340441699442; 293.726764975073; 1957.62557077626; 18345600; 0.209667950188188; 0.212930784377878; 0.604814068911827; 0.937350563262696; 0.313783218055011; 1330.99831331157; 18345741.4703196; 0.633445807243591; 1.91804831975127; 2.35409049574099; 0.732689201831818; -1.5344934463501; 101325; 18349200; 141.39777949085; 772.833011287532; 799.874159094406; 389.961821673668; 288.120548614084; 290.80814581048; 299.285752178871; 293.602726348459; 1975.8904109589; 18349200; 0.1779145265687; 0.17977096671111; 0.599980407789962; 0.970516826191994; 0.313594941202908; 1331.26012347496; ...(+15156 chars)], weaDat_wea_verboseRead=1, weaDat_wea_offset=0, weaDat_wea_startTime=0, weaDat_wea_timeEvents=1, sin_X=[0.01; 0.99], sin_p=101325, sin_T=285.15, vav1_vav_sta_default_p=101325, vav1_vav_sta_default_T=293.15, vav1_vav_sta_default_X=[0.01; 0.99], vav1_vav_riseTime=120, vav1_vav_y_start=1, vav1_vav_filter_gain=1, vav1_vav_filter_A_ripple=0.5, vav1_vav_filter_f_min=0, vav1_vav_filter_normalize368=1, vav1_vav_filter_x_start=[0; 0], vav1_vav_filter_u_nominal=1, vav1_vav_use_deltaM=1, vav1_vav_deltaM=0.3, vav1_vav_roundDuct=0, vav1_vav_ReC=4000, vav1_vav_a=-1.51, vav1_vav_b=9.45, vav1_vav_yL=0.166666666666667, vav1_vav_yU=0.611111111111111, vav1_vav_k1=0.45, vav1_vav_l=0.0001, vav1_vav_l2=0.01, vav1_vav_deltax=0.02, vav1_vav_y_min=0.02, vav1_terHea_bal1_preDro_s384=101325, vav1_terHea_bal1_preDro_s385=293.15, vav1_terHea_bal1_preDro_s386=[0.01; 0.99], vav1_terHea_bal2_preDro_s387=300000, vav1_terHea_bal2_preDro_s388=293.15, vav1_terHea_delta=0.001, vav1_terHea_T_a1_nominal=289.85, vav1_terHea_T_a2_nominal=355.35, vav1_terHea_r_nominal=0.666666666666667, vav1_terHea_hA_n_w=0.85, vav1_terHea_hA_n_a=0.8, vav1_terHea_hA_T0_w=293.15, vav1_terHea_hA_T0_a=293.15, vav1_sinTer_X=1, vav1_sinTer_p=300000, vav1_sinTer_T=293.15, vav1_souTer_X=1, vav1_souTer_m_flow=0, vav1_souTer_T=323.15, VSup1_T_start=293.15, VSup1_p_start=101325, VSup1_X_start=[0.01; 0.99], TDisVAV1_T_start=293.15, TDisVAV1_TAmb=293.15, TDisVAV1_tauHeaTra=1200, zer_k=0, vav2_vav_sta_default_p=101325, vav2_vav_sta_default_T=293.15, vav2_vav_sta_default_X=[0.01; 0.99], vav2_vav_riseTime=120, vav2_vav_y_start=1, vav2_vav_filter_gain=1, vav2_vav_filter_A_ripple=0.5, vav2_vav_filter_f_min=0, vav2_vav_filter_normalize418=1, vav2_vav_filter_x_start=[0; 0], vav2_vav_filter_u_nominal=1, vav2_vav_use_deltaM=1, vav2_vav_deltaM=0.3, vav2_vav_roundDuct=0, vav2_vav_ReC=4000, vav2_vav_a=-1.51, vav2_vav_b=9.45, vav2_vav_yL=0.166666666666667, vav2_vav_yU=0.611111111111111, vav2_vav_k1=0.45, vav2_vav_l=0.0001, vav2_vav_l2=0.01, vav2_vav_deltax=0.02, vav2_vav_y_min=0.02, vav2_terHea_bal1_preDro_s434=101325, vav2_terHea_bal1_preDro_s435=293.15, vav2_terHea_bal1_preDro_s436=[0.01; 0.99], vav2_terHea_bal2_preDro_s437=300000, vav2_terHea_bal2_preDro_s438=293.15, vav2_terHea_delta=0.001, vav2_terHea_T_a1_nominal=289.85, vav2_terHea_T_a2_nominal=355.35, vav2_terHea_r_nominal=0.666666666666667, vav2_terHea_hA_n_w=0.85, vav2_terHea_hA_n_a=0.8, vav2_terHea_hA_T0_w=293.15, vav2_terHea_hA_T0_a=293.15, vav2_sinTer_X=1, vav2_sinTer_p=300000, vav2_sinTer_T=293.15, vav2_souTer_X=1, vav2_souTer_m_flow=0, vav2_souTer_T=323.15, TDisVAV2_T_start=293.15, TDisVAV2_TAmb=293.15, TDisVAV2_tauHeaTra=1200, VSup2_T_start=293.15, VSup2_p_start=101325, VSup2_X_start=[0.01; 0.99], zon2_S_=0, zon2_E_=-1.5707963267949, zon2_W_=1.5707963267949, zon2_N_=3.14159265358979, zon2_matExtWal_absIR_a=0.9, zon2_matExtWal_absIR_b=0.9, zon2_matExtWal_absSol_a=0.6, zon2_matExtWal_absSol_b=0.6, zon2_matExtWal_roughness_467=3, zon2_matFlo_absIR_a=0.9, zon2_matFlo_absIR_b=0.9, zon2_matFlo_absSol_a=0.6, zon2_matFlo_absSol_b=0.6, zon2_matFlo_roughness_a=3, zon2_roof_absIR_a=0.9, zon2_roof_absIR_b=0.9, zon2_roof_absSol_a=0.6, zon2_roof_absSol_b=0.6, zon2_roof_roughness_a=3, zon2_window600_glass_1__x=0.003175, zon2_window600_glass_1__k=1.06, zon2_window600_glass_1__t480=0.86156, zon2_window600_glass_1__r481=0.0434, zon2_window600_glass_1__r482=0.0434, zon2_window600_glass_1__t483=0, zon2_window600_glass_1__a484=0.9, zon2_window600_glass_1__a485=0.9, zon2_window600_glass_2__x=0.003175, zon2_window600_glass_2__k=1.06, zon2_window600_glass_2__t488=0.86156, zon2_window600_glass_2__r489=0.0434, zon2_window600_glass_2__r490=0.0434, zon2_window600_glass_2__t491=0, zon2_window600_glass_2__a492=0.9, zon2_window600_glass_2__a493=0.9, zon2_window600_gas_1__x=0.013, zon2_window600_gas_1__a_k=0.002873, zon2_window600_gas_1__b_k=7.76e-05, zon2_window600_gas_1__a_m497=3.723e-06, zon2_window600_gas_1__b_m498=4.94e-08, zon2_window600_gas_1__a_c=1002.737, zon2_window600_gas_1__b_c=0.012324, zon2_window600_gas_1__MM=0.02897, zon2_window600_gas_1__P0=101325, zon2_window600_shade_tauS503=0.1, zon2_window600_shade_tauS504=0.1, zon2_window600_shade_rhoS505=0.8, zon2_window600_shade_rhoS506=0.8, zon2_window600_shade_absI507=0.84, zon2_window600_shade_absI508=0.84, zon2_window600_shade_tauI509=0, zon2_window600_shade_tauI510=0, zon2_window600_UFra=3, zon2_window600_absIRFra=0.8, zon2_window600_absSolFra=0.5, zon2_soi_A=48, zon2_soi_T_a_start=283.15, zon2_soi_T_b_start=283.75, zon2_roo_datConExt_1__bou517=1, zon2_roo_datConExt_1__A=48, zon2_roo_datConExt_2__bou519=1, zon2_roo_datConExt_2__A=16.2, zon2_roo_datConExt_3__bou521=1, zon2_roo_datConExt_3__A=16.2, zon2_roo_datConExt_4__bou523=1, zon2_roo_datConExt_4__A=21.6, zon2_roo_datConExtWin_1__525=1, zon2_roo_datConExtWin_1__526=21.6, zon2_roo_datConExtWin_1__527=2, zon2_roo_datConExtWin_1__528=6, zon2_roo_datConExtWin_1__529=0.001, zon2_roo_datConExtWin_1__530=0, zon2_roo_datConExtWin_1__531=0, zon2_roo_datConExtWin_1__532=0, zon2_roo_datConExtWin_1__533=0, zon2_roo_datConExtWin_1__534=0, zon2_roo_datConPar_1__azi=0, zon2_roo_datConPar_1__bou536=1, zon2_roo_datConPar_1__A=0, zon2_roo_datConBou_1__azi=0, zon2_roo_datConBou_1__bou539=1, zon2_roo_datConBou_1__A=48, zon2_roo_surBou_1__A=0, zon2_roo_surBou_1__absIR=0.84, zon2_roo_surBou_1__absSol=0.84, zon2_roo_surBou_1__bounda544=1, zon2_roo_dummyCon_absIR_a=0.9, zon2_roo_dummyCon_absIR_b=0.9, zon2_roo_dummyCon_absSol_547=0.5, zon2_roo_dummyCon_absSol_548=0.5, zon2_roo_dummyCon_roughne549=3, zon2_roo_dummyGlaSys_glas550=0.003, zon2_roo_dummyGlaSys_glas551=1, zon2_roo_dummyGlaSys_glas552=0.834, zon2_roo_dummyGlaSys_glas553=0.075, zon2_roo_dummyGlaSys_glas554=0.075, zon2_roo_dummyGlaSys_glas555=0, zon2_roo_dummyGlaSys_glas556=0.84, zon2_roo_dummyGlaSys_glas557=0.84, zon2_roo_dummyGlaSys_gas_558=-1, zon2_roo_dummyGlaSys_gas_559=0.002873, zon2_roo_dummyGlaSys_gas_560=7.76e-05, zon2_roo_dummyGlaSys_gas_561=3.723e-06, zon2_roo_dummyGlaSys_gas_562=4.94e-08, zon2_roo_dummyGlaSys_gas_563=1002.737, zon2_roo_dummyGlaSys_gas_564=0.012324, zon2_roo_dummyGlaSys_gas_565=0.02897, zon2_roo_dummyGlaSys_gas_566=101325, zon2_roo_dummyGlaSys_shad567=0.1, zon2_roo_dummyGlaSys_shad568=0.1, zon2_roo_dummyGlaSys_shad569=0.8, zon2_roo_dummyGlaSys_shad570=0.8, zon2_roo_dummyGlaSys_shad571=0.84, zon2_roo_dummyGlaSys_shad572=0.84, zon2_roo_dummyGlaSys_shad573=0, zon2_roo_dummyGlaSys_shad574=0, zon2_roo_dummyGlaSys_UFra=3, zon2_roo_dummyGlaSys_absI576=0.8, zon2_roo_dummyGlaSys_absS577=0.5, zon2_roo_AFlo=48, zon2_roo_hRoo=2.7, zon2_roo_conExtWin_1__gla580=0, zon2_roo_conExtWin_1__win581=1, zon2_roo_conExtWin_1__win582=3, zon2_roo_conExtWin_1__win583=331.4, zon2_roo_conExtWin_1__win584=1, zon2_roo_hIntFixed=3, zon2_roo_hExtFixed=10, zon2_roo_bouConExt_HDifTi587=0.2, zon2_roo_bouConExt_HDifTi588=1, zon2_roo_bouConExt_HDifTi589=1, zon2_roo_bouConExt_HDifTi590=0.2, zon2_roo_bouConExt_HDifTi591=1, zon2_roo_bouConExt_HDifTi592=1, zon2_roo_bouConExt_HDifTi593=0.2, zon2_roo_bouConExt_HDifTi594=1, zon2_roo_bouConExt_HDifTi595=1, zon2_roo_bouConExt_HDifTi596=0.2, zon2_roo_bouConExt_HDifTi597=1, zon2_roo_bouConExt_HDifTi598=1, zon2_roo_bouConExtWin_con599=0, zon2_roo_bouConExtWin_con600=0, zon2_roo_bouConExtWin_HDi601=0.2, zon2_roo_bouConExtWin_HDi602=1, zon2_roo_bouConExtWin_HDi603=1, zon2_roo_bouConExtWin_con604=293.15, zon2_roo_air_datConExtWin605=0, zon2_roo_air_datConExtWin606=0, zon2_roo_air_dummyCon_abs607=0.9, zon2_roo_air_dummyCon_abs608=0.9, zon2_roo_air_dummyCon_abs609=0.5, zon2_roo_air_dummyCon_abs610=0.5, zon2_roo_air_dummyCon_rou611=3, zon2_roo_air_dummyGlaSys_612=0.003, zon2_roo_air_dummyGlaSys_613=1, zon2_roo_air_dummyGlaSys_614=0.834, zon2_roo_air_dummyGlaSys_615=0.075, zon2_roo_air_dummyGlaSys_616=0.075, zon2_roo_air_dummyGlaSys_617=0, zon2_roo_air_dummyGlaSys_618=0.84, zon2_roo_air_dummyGlaSys_619=0.84, zon2_roo_air_dummyGlaSys_620=-1, zon2_roo_air_dummyGlaSys_621=0.002873, zon2_roo_air_dummyGlaSys_622=7.76e-05, zon2_roo_air_dummyGlaSys_623=3.723e-06, zon2_roo_air_dummyGlaSys_624=4.94e-08, zon2_roo_air_dummyGlaSys_625=1002.737, zon2_roo_air_dummyGlaSys_626=0.012324, zon2_roo_air_dummyGlaSys_627=0.02897, zon2_roo_air_dummyGlaSys_628=101325, zon2_roo_air_dummyGlaSys_629=0.1, zon2_roo_air_dummyGlaSys_630=0.1, zon2_roo_air_dummyGlaSys_631=0.8, zon2_roo_air_dummyGlaSys_632=0.8, zon2_roo_air_dummyGlaSys_633=0.84, zon2_roo_air_dummyGlaSys_634=0.84, zon2_roo_air_dummyGlaSys_635=0, zon2_roo_air_dummyGlaSys_636=0, zon2_roo_air_dummyGlaSys_637=3, zon2_roo_air_dummyGlaSys_638=0.8, zon2_roo_air_dummyGlaSys_639=0.5, zon2_roo_solRadExc_datCon640=0, zon2_roo_solRadExc_datCon641=0, zon2_roo_solRadExc_dummyC642=0.9, zon2_roo_solRadExc_dummyC643=0.9, zon2_roo_solRadExc_dummyC644=0.5, zon2_roo_solRadExc_dummyC645=0.5, zon2_roo_solRadExc_dummyC646=3, zon2_roo_solRadExc_dummyG647=0.003, zon2_roo_solRadExc_dummyG648=1, zon2_roo_solRadExc_dummyG649=0.834, zon2_roo_solRadExc_dummyG650=0.075, zon2_roo_solRadExc_dummyG651=0.075, zon2_roo_solRadExc_dummyG652=0, zon2_roo_solRadExc_dummyG653=0.84, zon2_roo_solRadExc_dummyG654=0.84, zon2_roo_solRadExc_dummyG655=-1, zon2_roo_solRadExc_dummyG656=0.002873, zon2_roo_solRadExc_dummyG657=7.76e-05, zon2_roo_solRadExc_dummyG658=3.723e-06, zon2_roo_solRadExc_dummyG659=4.94e-08, zon2_roo_solRadExc_dummyG660=1002.737, zon2_roo_solRadExc_dummyG661=0.012324, zon2_roo_solRadExc_dummyG662=0.02897, zon2_roo_solRadExc_dummyG663=101325, zon2_roo_solRadExc_dummyG664=0.1, zon2_roo_solRadExc_dummyG665=0.1, zon2_roo_solRadExc_dummyG666=0.8, zon2_roo_solRadExc_dummyG667=0.8, zon2_roo_solRadExc_dummyG668=0.84, zon2_roo_solRadExc_dummyG669=0.84, zon2_roo_solRadExc_dummyG670=0, zon2_roo_solRadExc_dummyG671=0, zon2_roo_solRadExc_dummyG672=3, zon2_roo_solRadExc_dummyG673=0.8, zon2_roo_solRadExc_dummyG674=0.5, zon2_roo_irRadGai_datConE675=0, zon2_roo_irRadGai_datConE676=0, zon2_roo_irRadGai_dummyCo677=0.9, zon2_roo_irRadGai_dummyCo678=0.9, zon2_roo_irRadGai_dummyCo679=0.5, zon2_roo_irRadGai_dummyCo680=0.5, zon2_roo_irRadGai_dummyCo681=3, zon2_roo_irRadGai_dummyGl682=0.003, zon2_roo_irRadGai_dummyGl683=1, zon2_roo_irRadGai_dummyGl684=0.834, zon2_roo_irRadGai_dummyGl685=0.075, zon2_roo_irRadGai_dummyGl686=0.075, zon2_roo_irRadGai_dummyGl687=0, zon2_roo_irRadGai_dummyGl688=0.84, zon2_roo_irRadGai_dummyGl689=0.84, zon2_roo_irRadGai_dummyGl690=-1, zon2_roo_irRadGai_dummyGl691=0.002873, zon2_roo_irRadGai_dummyGl692=7.76e-05, zon2_roo_irRadGai_dummyGl693=3.723e-06, zon2_roo_irRadGai_dummyGl694=4.94e-08, zon2_roo_irRadGai_dummyGl695=1002.737, zon2_roo_irRadGai_dummyGl696=0.012324, zon2_roo_irRadGai_dummyGl697=0.02897, zon2_roo_irRadGai_dummyGl698=101325, zon2_roo_irRadGai_dummyGl699=0.1, zon2_roo_irRadGai_dummyGl700=0.1, zon2_roo_irRadGai_dummyGl701=0.8, zon2_roo_irRadGai_dummyGl702=0.8, zon2_roo_irRadGai_dummyGl703=0.84, zon2_roo_irRadGai_dummyGl704=0.84, zon2_roo_irRadGai_dummyGl705=0, zon2_roo_irRadGai_dummyGl706=0, zon2_roo_irRadGai_dummyGl707=3, zon2_roo_irRadGai_dummyGl708=0.8, zon2_roo_irRadGai_dummyGl709=0.5, zon2_roo_irRadExc_datConE710=0, zon2_roo_irRadExc_datConE711=0, zon2_roo_irRadExc_dummyCo712=0.9, zon2_roo_irRadExc_dummyCo713=0.9, zon2_roo_irRadExc_dummyCo714=0.5, zon2_roo_irRadExc_dummyCo715=0.5, zon2_roo_irRadExc_dummyCo716=3, zon2_roo_irRadExc_dummyGl717=0.003, zon2_roo_irRadExc_dummyGl718=1, zon2_roo_irRadExc_dummyGl719=0.834, zon2_roo_irRadExc_dummyGl720=0.075, zon2_roo_irRadExc_dummyGl721=0.075, zon2_roo_irRadExc_dummyGl722=0, zon2_roo_irRadExc_dummyGl723=0.84, zon2_roo_irRadExc_dummyGl724=0.84, zon2_roo_irRadExc_dummyGl725=-1, zon2_roo_irRadExc_dummyGl726=0.002873, zon2_roo_irRadExc_dummyGl727=7.76e-05, zon2_roo_irRadExc_dummyGl728=3.723e-06, zon2_roo_irRadExc_dummyGl729=4.94e-08, zon2_roo_irRadExc_dummyGl730=1002.737, zon2_roo_irRadExc_dummyGl731=0.012324, zon2_roo_irRadExc_dummyGl732=0.02897, zon2_roo_irRadExc_dummyGl733=101325, zon2_roo_irRadExc_dummyGl734=0.1, zon2_roo_irRadExc_dummyGl735=0.1, zon2_roo_irRadExc_dummyGl736=0.8, zon2_roo_irRadExc_dummyGl737=0.8, zon2_roo_irRadExc_dummyGl738=0.84, zon2_roo_irRadExc_dummyGl739=0.84, zon2_roo_irRadExc_dummyGl740=0, zon2_roo_irRadExc_dummyGl741=0, zon2_roo_irRadExc_dummyGl742=3, zon2_roo_irRadExc_dummyGl743=0.8, zon2_roo_irRadExc_dummyGl744=0.5, zon2_roo_irRadExc_T0=293.15, zon2_roo_radTem_datConExt746=0, zon2_roo_radTem_datConExt747=0, zon2_roo_radTem_dummyCon_748=0.9, zon2_roo_radTem_dummyCon_749=0.9, zon2_roo_radTem_dummyCon_750=0.5, zon2_roo_radTem_dummyCon_751=0.5, zon2_roo_radTem_dummyCon_752=3, zon2_roo_radTem_dummyGlaS753=0.003, zon2_roo_radTem_dummyGlaS754=1, zon2_roo_radTem_dummyGlaS755=0.834, zon2_roo_radTem_dummyGlaS756=0.075, zon2_roo_radTem_dummyGlaS757=0.075, zon2_roo_radTem_dummyGlaS758=0, zon2_roo_radTem_dummyGlaS759=0.84, zon2_roo_radTem_dummyGlaS760=0.84, zon2_roo_radTem_dummyGlaS761=-1, zon2_roo_radTem_dummyGlaS762=0.002873, zon2_roo_radTem_dummyGlaS763=7.76e-05, zon2_roo_radTem_dummyGlaS764=3.723e-06, zon2_roo_radTem_dummyGlaS765=4.94e-08, zon2_roo_radTem_dummyGlaS766=1002.737, zon2_roo_radTem_dummyGlaS767=0.012324, zon2_roo_radTem_dummyGlaS768=0.02897, zon2_roo_radTem_dummyGlaS769=101325, zon2_roo_radTem_dummyGlaS770=0.1, zon2_roo_radTem_dummyGlaS771=0.1, zon2_roo_radTem_dummyGlaS772=0.8, zon2_roo_radTem_dummyGlaS773=0.8, zon2_roo_radTem_dummyGlaS774=0.84, zon2_roo_radTem_dummyGlaS775=0.84, zon2_roo_radTem_dummyGlaS776=0, zon2_roo_radTem_dummyGlaS777=0, zon2_roo_radTem_dummyGlaS778=3, zon2_roo_radTem_dummyGlaS779=0.8, zon2_roo_radTem_dummyGlaS780=0.5, zon2_roo_add_k1=1, zon2_roo_add_k2=1, zon2_roo_sumJFroWin_1__k=1, zon2_roo_p_start=101325, zon2_roo_T_start=293.15, zon2_roo_X_start=[0.01; 0.99], zon2_qConGai_flow_k=4, zon2_qRadGai_flow_k=6, zon2_qLatGai_flow_k=2, zon2_TSoi_1__T=283.15, zon2_sinInf_m_flow=0, zon2_sinInf_x_pTphi_p=101325, zon2_InfiltrationRate_k=0.018, zon2_souInf_m_flow=0, zon2_souInf_x_pTphi_p=101325, zon2_intLoad_table=[0; 0.1; 28800; 0.1; 28800; 1; 64800; 1; 64800; 0.1; 86400; 0.1], zon2_intLoad_verboseRead=1, zon2_intLoad_columns=2, zon2_intLoad_offset=0, zon2_intLoad_startTime=0, zon2_intLoad_timeEvents=1, zon1_roo_conExtWin_1__win802=293.15, zon1_roo_conExtWin_1__win803=293.15, zon1_roo_conExtWin_1__win804=293.15, zon2_roo_conExtWin_1__win805=293.15, zon2_roo_conExtWin_1__win806=293.15, zon2_roo_conExtWin_1__win807=293.15}
      mask prompts: zon1_S_ "zon1.S_"; zon1_E_ "zon1.E_"; zon1_W_ "zon1.W_"; zon1_N_ "zon1.N_"; zon1_matExtWal_absIR_a "zon1.matExtWal.absIR_a"; zon1_matExtWal_absIR_b "zon1.matExtWal.absIR_b"; zon1_matExtWal_absSol_a "zon1.matExtWal.absSol_a"; zon1_matExtWal_absSol_b "zon1.matExtWal.absSol_b"; zon1_matExtWal_roughness_10 "zon1.matExtWal.roughness_a"; zon1_matFlo_absIR_a "zon1.matFlo.absIR_a"; zon1_matFlo_absIR_b "zon1.matFlo.absIR_b"; zon1_matFlo_absSol_a "zon1.matFlo.absSol_a"; zon1_matFlo_absSol_b "zon1.matFlo.absSol_b"; zon1_matFlo_roughness_a "zon1.matFlo.roughness_a"; zon1_roof_absIR_a "zon1.roof.absIR_a"; zon1_roof_absIR_b "zon1.roof.absIR_b"; zon1_roof_absSol_a "zon1.roof.absSol_a"; zon1_roof_absSol_b "zon1.roof.absSol_b"; zon1_roof_roughness_a "zon1.roof.roughness_a"; zon1_window600_glass_1__x "zon1.window600.glass[1].x"; zon1_window600_glass_1__k "zon1.window600.glass[1].k"; zon1_window600_glass_1__t23 "zon1.window600.glass[1].tauSol"; zon1_window600_glass_1__r24 "zon1.window600.glass[1].rhoSol_a"; zon1_window600_glass_1__r25 "zon1.window600.glass[1].rhoSol_b"; zon1_window600_glass_1__t26 "zon1.window600.glass[1].tauIR"; zon1_window600_glass_1__a27 "zon1.window600.glass[1].absIR_a"; zon1_window600_glass_1__a28 "zon1.window600.glass[1].absIR_b"; zon1_window600_glass_2__x "zon1.window600.glass[2].x"; zon1_window600_glass_2__k "zon1.window600.glass[2].k"; zon1_window600_glass_2__t31 "zon1.window600.glass[2].tauSol"; zon1_window600_glass_2__r32 "zon1.window600.glass[2].rhoSol_a"; zon1_window600_glass_2__r33 "zon1.window600.glass[2].rhoSol_b"; zon1_window600_glass_2__t34 "zon1.window600.glass[2].tauIR"; zon1_window600_glass_2__a35 "zon1.window600.glass[2].absIR_a"; zon1_window600_glass_2__a36 "zon1.window600.glass[2].absIR_b"; zon1_window600_gas_1__x "zon1.window600.gas[1].x"; zon1_window600_gas_1__a_k "zon1.window600.gas[1].a_k"; zon1_window600_gas_1__b_k "zon1.window600.gas[1].b_k"; zon1_window600_gas_1__a_m40 "zon1.window600.gas[1].a_mu"; zon1_window600_gas_1__b_m41 "zon1.window600.gas[1].b_mu"; zon1_window600_gas_1__a_c "zon1.window600.gas[1].a_c"; zon1_window600_gas_1__b_c "zon1.window600.gas[1].b_c"; zon1_window600_gas_1__MM "zon1.window600.gas[1].MM"; zon1_window600_gas_1__P0 "zon1.window600.gas[1].P0"; zon1_window600_shade_tauS46 "zon1.window600.shade.tauSol_a"; zon1_window600_shade_tauS47 "zon1.window600.shade.tauSol_b"; zon1_window600_shade_rhoS48 "zon1.window600.shade.rhoSol_a"; zon1_window600_shade_rhoS49 "zon1.window600.shade.rhoSol_b"; zon1_window600_shade_absI50 "zon1.window600.shade.absIR_a"; zon1_window600_shade_absI51 "zon1.window600.shade.absIR_b"; zon1_window600_shade_tauI52 "zon1.window600.shade.tauIR_a"; zon1_window600_shade_tauI53 "zon1.window600.shade.tauIR_b"; zon1_window600_UFra "zon1.window600.UFra"; zon1_window600_absIRFra "zon1.window600.absIRFra"; zon1_window600_absSolFra "zon1.window600.absSolFra"; zon1_soi_A "zon1.soi.A"; zon1_soi_T_a_start "zon1.soi.T_a_start"; zon1_soi_T_b_start "zon1.soi.T_b_start"; zon1_roo_datConExt_1__bou60 "zon1.roo.datConExt[1].boundaryCondition"; zon1_roo_datConExt_1__A "zon1.roo.datConExt[1].A"; zon1_roo_datConExt_2__bou62 "zon1.roo.datConExt[2].boundaryCondition"; zon1_roo_datConExt_2__A "zon1.roo.datConExt[2].A"; zon1_roo_datConExt_3__bou64 "zon1.roo.datConExt[3].boundaryCondition"; zon1_roo_datConExt_3__A "zon1.roo.datConExt[3].A"; zon1_roo_datConExt_4__bou66 "zon1.roo.datConExt[4].boundaryCondition"; zon1_roo_datConExt_4__A "zon1.roo.datConExt[4].A"; zon1_roo_datConExtWin_1__68 "zon1.roo.datConExtWin[1].boundaryCondition"; zon1_roo_datConExtWin_1__69 "zon1.roo.datConExtWin[1].A"; zon1_roo_datConExtWin_1__70 "zon1.roo.datConExtWin[1].hWin"; zon1_roo_datConExtWin_1__71 "zon1.roo.datConExtWin[1].wWin"; zon1_roo_datConExtWin_1__72 "zon1.roo.datConExtWin[1].fFra"; zon1_roo_datConExtWin_1__73 "zon1.roo.datConExtWin[1].ove.wL"; zon1_roo_datConExtWin_1__74 "zon1.roo.datConExtWin[1].ove.wR"; zon1_roo_datConExtWin_1__75 "zon1.roo.datConExtWin[1].ove.gap"; zon1_roo_datConExtWin_1__76 "zon1.roo.datConExtWin[1].sidFin.h"; zon1_roo_datConExtWin_1__77 "zon1.roo.datConExtWin[1].sidFin.gap"; zon1_roo_datConPar_1__azi "zon1.roo.datConPar[1].azi"; zon1_roo_datConPar_1__bou79 "zon1.roo.datConPar[1].boundaryCondition"; zon1_roo_datConPar_1__A "zon1.roo.datConPar[1].A"; zon1_roo_datConBou_1__azi "zon1.roo.datConBou[1].azi"; zon1_roo_datConBou_1__bou82 "zon1.roo.datConBou[1].boundaryCondition"; zon1_roo_datConBou_1__A "zon1.roo.datConBou[1].A"; zon1_roo_surBou_1__A "zon1.roo.surBou[1].A"; zon1_roo_surBou_1__absIR "zon1.roo.surBou[1].absIR"; zon1_roo_surBou_1__absSol "zon1.roo.surBou[1].absSol"; zon1_roo_surBou_1__bounda87 "zon1.roo.surBou[1].boundaryCondition"; zon1_roo_dummyCon_absIR_a "zon1.roo.dummyCon.absIR_a"; zon1_roo_dummyCon_absIR_b "zon1.roo.dummyCon.absIR_b"; zon1_roo_dummyCon_absSol_90 "zon1.roo.dummyCon.absSol_a"; zon1_roo_dummyCon_absSol_91 "zon1.roo.dummyCon.absSol_b"; zon1_roo_dummyCon_roughne92 "zon1.roo.dummyCon.roughness_a"; zon1_roo_dummyGlaSys_glas93 "zon1.roo.dummyGlaSys.glass[1].x"; zon1_roo_dummyGlaSys_glas94 "zon1.roo.dummyGlaSys.glass[1].k"; zon1_roo_dummyGlaSys_glas95 "zon1.roo.dummyGlaSys.glass[1].tauSol"; zon1_roo_dummyGlaSys_glas96 "zon1.roo.dummyGlaSys.glass[1].rhoSol_a"; zon1_roo_dummyGlaSys_glas97 "zon1.roo.dummyGlaSys.glass[1].rhoSol_b"; zon1_roo_dummyGlaSys_glas98 "zon1.roo.dummyGlaSys.glass[1].tauIR"; zon1_roo_dummyGlaSys_glas99 "zon1.roo.dummyGlaSys.glass[1].absIR_a"; zon1_roo_dummyGlaSys_glas100 "zon1.roo.dummyGlaSys.glass[1].absIR_b"; zon1_roo_dummyGlaSys_gas_101 "zon1.roo.dummyGlaSys.gas[1].x"; zon1_roo_dummyGlaSys_gas_102 "zon1.roo.dummyGlaSys.gas[1].a_k"; zon1_roo_dummyGlaSys_gas_103 "zon1.roo.dummyGlaSys.gas[1].b_k"; zon1_roo_dummyGlaSys_gas_104 "zon1.roo.dummyGlaSys.gas[1].a_mu"; zon1_roo_dummyGlaSys_gas_105 "zon1.roo.dummyGlaSys.gas[1].b_mu"; zon1_roo_dummyGlaSys_gas_106 "zon1.roo.dummyGlaSys.gas[1].a_c"; zon1_roo_dummyGlaSys_gas_107 "zon1.roo.dummyGlaSys.gas[1].b_c"; zon1_roo_dummyGlaSys_gas_108 "zon1.roo.dummyGlaSys.gas[1].MM"; zon1_roo_dummyGlaSys_gas_109 "zon1.roo.dummyGlaSys.gas[1].P0"; zon1_roo_dummyGlaSys_shad110 "zon1.roo.dummyGlaSys.shade.tauSol_a"; zon1_roo_dummyGlaSys_shad111 "zon1.roo.dummyGlaSys.shade.tauSol_b"; zon1_roo_dummyGlaSys_shad112 "zon1.roo.dummyGlaSys.shade.rhoSol_a"; zon1_roo_dummyGlaSys_shad113 "zon1.roo.dummyGlaSys.shade.rhoSol_b"; zon1_roo_dummyGlaSys_shad114 "zon1.roo.dummyGlaSys.shade.absIR_a"; zon1_roo_dummyGlaSys_shad115 "zon1.roo.dummyGlaSys.shade.absIR_b"; zon1_roo_dummyGlaSys_shad116 "zon1.roo.dummyGlaSys.shade.tauIR_a"; zon1_roo_dummyGlaSys_shad117 "zon1.roo.dummyGlaSys.shade.tauIR_b"; zon1_roo_dummyGlaSys_UFra "zon1.roo.dummyGlaSys.UFra"; zon1_roo_dummyGlaSys_absI119 "zon1.roo.dummyGlaSys.absIRFra"; zon1_roo_dummyGlaSys_absS120 "zon1.roo.dummyGlaSys.absSolFra"; zon1_roo_AFlo "zon1.roo.AFlo"; zon1_roo_hRoo "zon1.roo.hRoo"; zon1_roo_conExtWin_1__gla123 "zon1.roo.conExtWin[1].glaSys.haveControllableWindow"; zon1_roo_conExtWin_1__win124 "zon1.roo.conExtWin[1].win.matGla.k"; zon1_roo_conExtWin_1__win125 "zon1.roo.conExtWin[1].win.matGla.nStaRef"; zon1_roo_conExtWin_1__win126 "zon1.roo.conExtWin[1].win.matGla.piRef"; zon1_roo_conExtWin_1__win127 "zon1.roo.conExtWin[1].win.matGla.nStaReal"; zon1_roo_hIntFixed "zon1.roo.hIntFixed"; zon1_roo_hExtFixed "zon1.roo.hExtFixed"; zon1_roo_bouConExt_HDifTi130 "zon1.roo.bouConExt.HDifTil[1].rho"; zon1_roo_bouConExt_HDifTi131 "zon1.roo.bouConExt.HDifTil[1].add.k1"; zon1_roo_bouConExt_HDifTi132 "zon1.roo.bouConExt.HDifTil[1].add.k2"; zon1_roo_bouConExt_HDifTi133 "zon1.roo.bouConExt.HDifTil[2].rho"; zon1_roo_bouConExt_HDifTi134 "zon1.roo.bouConExt.HDifTil[2].add.k1"; zon1_roo_bouConExt_HDifTi135 "zon1.roo.bouConExt.HDifTil[2].add.k2"; zon1_roo_bouConExt_HDifTi136 "zon1.roo.bouConExt.HDifTil[3].rho"; zon1_roo_bouConExt_HDifTi137 "zon1.roo.bouConExt.HDifTil[3].add.k1"; zon1_roo_bouConExt_HDifTi138 "zon1.roo.bouConExt.HDifTil[3].add.k2"; zon1_roo_bouConExt_HDifTi139 "zon1.roo.bouConExt.HDifTil[4].rho"; zon1_roo_bouConExt_HDifTi140 "zon1.roo.bouConExt.HDifTil[4].add.k1"; zon1_roo_bouConExt_HDifTi141 "zon1.roo.bouConExt.HDifTil[4].add.k2"; zon1_roo_bouConExtWin_con142 "zon1.roo.bouConExtWin.conPar[1].ove.dep"; zon1_roo_bouConExtWin_con143 "zon1.roo.bouConExtWin.conPar[1].sidFin.dep"; zon1_roo_bouConExtWin_HDi144 "zon1.roo.bouConExtWin.HDifTil[1].rho"; zon1_roo_bouConExtWin_HDi145 "zon1.roo.bouConExtWin.HDifTil[1].add.k1"; zon1_roo_bouConExtWin_HDi146 "zon1.roo.bouConExtWin.HDifTil[1].add.k2"; zon1_roo_bouConExtWin_con147 "zon1.roo.bouConExtWin.conExtWin[1].radOut.T0"; zon1_roo_air_datConExtWin148 "zon1.roo.air.datConExtWin[1].ove.dep"; zon1_roo_air_datConExtWin149 "zon1.roo.air.datConExtWin[1].sidFin.dep"; zon1_roo_air_dummyCon_abs150 "zon1.roo.air.dummyCon.absIR_a"; zon1_roo_air_dummyCon_abs151 "zon1.roo.air.dummyCon.absIR_b"; zon1_roo_air_dummyCon_abs152 "zon1.roo.air.dummyCon.absSol_a"; zon1_roo_air_dummyCon_abs153 "zon1.roo.air.dummyCon.absSol_b"; zon1_roo_air_dummyCon_rou154 "zon1.roo.air.dummyCon.roughness_a"; zon1_roo_air_dummyGlaSys_155 "zon1.roo.air.dummyGlaSys.glass[1].x"; zon1_roo_air_dummyGlaSys_156 "zon1.roo.air.dummyGlaSys.glass[1].k"; zon1_roo_air_dummyGlaSys_157 "zon1.roo.air.dummyGlaSys.glass[1].tauSol"; zon1_roo_air_dummyGlaSys_158 "zon1.roo.air.dummyGlaSys.glass[1].rhoSol_a"; zon1_roo_air_dummyGlaSys_159 "zon1.roo.air.dummyGlaSys.glass[1].rhoSol_b"; zon1_roo_air_dummyGlaSys_160 "zon1.roo.air.dummyGlaSys.glass[1].tauIR"; zon1_roo_air_dummyGlaSys_161 "zon1.roo.air.dummyGlaSys.glass[1].absIR_a"; zon1_roo_air_dummyGlaSys_162 "zon1.roo.air.dummyGlaSys.glass[1].absIR_b"; zon1_roo_air_dummyGlaSys_163 "zon1.roo.air.dummyGlaSys.gas[1].x"; zon1_roo_air_dummyGlaSys_164 "zon1.roo.air.dummyGlaSys.gas[1].a_k"; zon1_roo_air_dummyGlaSys_165 "zon1.roo.air.dummyGlaSys.gas[1].b_k"; zon1_roo_air_dummyGlaSys_166 "zon1.roo.air.dummyGlaSys.gas[1].a_mu"; zon1_roo_air_dummyGlaSys_167 "zon1.roo.air.dummyGlaSys.gas[1].b_mu"; zon1_roo_air_dummyGlaSys_168 "zon1.roo.air.dummyGlaSys.gas[1].a_c"; zon1_roo_air_dummyGlaSys_169 "zon1.roo.air.dummyGlaSys.gas[1].b_c"; zon1_roo_air_dummyGlaSys_170 "zon1.roo.air.dummyGlaSys.gas[1].MM"; zon1_roo_air_dummyGlaSys_171 "zon1.roo.air.dummyGlaSys.gas[1].P0"; zon1_roo_air_dummyGlaSys_172 "zon1.roo.air.dummyGlaSys.shade.tauSol_a"; zon1_roo_air_dummyGlaSys_173 "zon1.roo.air.dummyGlaSys.shade.tauSol_b"; zon1_roo_air_dummyGlaSys_174 "zon1.roo.air.dummyGlaSys.shade.rhoSol_a"; zon1_roo_air_dummyGlaSys_175 "zon1.roo.air.dummyGlaSys.shade.rhoSol_b"; zon1_roo_air_dummyGlaSys_176 "zon1.roo.air.dummyGlaSys.shade.absIR_a"; zon1_roo_air_dummyGlaSys_177 "zon1.roo.air.dummyGlaSys.shade.absIR_b"; zon1_roo_air_dummyGlaSys_178 "zon1.roo.air.dummyGlaSys.shade.tauIR_a"; zon1_roo_air_dummyGlaSys_179 "zon1.roo.air.dummyGlaSys.shade.tauIR_b"; zon1_roo_air_dummyGlaSys_180 "zon1.roo.air.dummyGlaSys.UFra"; zon1_roo_air_dummyGlaSys_181 "zon1.roo.air.dummyGlaSys.absIRFra"; zon1_roo_air_dummyGlaSys_182 "zon1.roo.air.dummyGlaSys.absSolFra"; zon1_roo_solRadExc_datCon183 "zon1.roo.solRadExc.datConExtWin[1].ove.dep"; zon1_roo_solRadExc_datCon184 "zon1.roo.solRadExc.datConExtWin[1].sidFin.dep"; zon1_roo_solRadExc_dummyC185 "zon1.roo.solRadExc.dummyCon.absIR_a"; zon1_roo_solRadExc_dummyC186 "zon1.roo.solRadExc.dummyCon.absIR_b"; zon1_roo_solRadExc_dummyC187 "zon1.roo.solRadExc.dummyCon.absSol_a"; zon1_roo_solRadExc_dummyC188 "zon1.roo.solRadExc.dummyCon.absSol_b"; zon1_roo_solRadExc_dummyC189 "zon1.roo.solRadExc.dummyCon.roughness_a"; zon1_roo_solRadExc_dummyG190 "zon1.roo.solRadExc.dummyGlaSys.glass[1].x"; zon1_roo_solRadExc_dummyG191 "zon1.roo.solRadExc.dummyGlaSys.glass[1].k"; zon1_roo_solRadExc_dummyG192 "zon1.roo.solRadExc.dummyGlaSys.glass[1].tauSol"; zon1_roo_solRadExc_dummyG193 "zon1.roo.solRadExc.dummyGlaSys.glass[1].rhoSol_a"; zon1_roo_solRadExc_dummyG194 "zon1.roo.solRadExc.dummyGlaSys.glass[1].rhoSol_b"; zon1_roo_solRadExc_dummyG195 "zon1.roo.solRadExc.dummyGlaSys.glass[1].tauIR"; zon1_roo_solRadExc_dummyG196 "zon1.roo.solRadExc.dummyGlaSys.glass[1].absIR_a"; zon1_roo_solRadExc_dummyG197 "zon1.roo.solRadExc.dummyGlaSys.glass[1].absIR_b"; zon1_roo_solRadExc_dummyG198 "zon1.roo.solRadExc.dummyGlaSys.gas[1].x"; zon1_roo_solRadExc_dummyG199 "zon1.roo.solRadExc.dummyGlaSys.gas[1].a_k"; zon1_roo_solRadExc_dummyG200 "zon1.roo.solRadExc.dummyGlaSys.gas[1].b_k"; zon1_roo_solRadExc_dummyG201 "zon1.roo.solRadExc.dummyGlaSys.gas[1].a_mu"; zon1_roo_solRadExc_dummyG202 "zon1.roo.solRadExc.dummyGlaSys.gas[1].b_mu"; zon1_roo_solRadExc_dummyG203 "zon1.roo.solRadExc.dummyGlaSys.gas[1].a_c"; zon1_roo_solRadExc_dummyG204 "zon1.roo.solRadExc.dummyGlaSys.gas[1].b_c"; zon1_roo_solRadExc_dummyG205 "zon1.roo.solRadExc.dummyGlaSys.gas[1].MM"; zon1_roo_solRadExc_dummyG206 "zon1.roo.solRadExc.dummyGlaSys.gas[1].P0"; zon1_roo_solRadExc_dummyG207 "zon1.roo.solRadExc.dummyGlaSys.shade.tauSol_a"; zon1_roo_solRadExc_dummyG208 "zon1.roo.solRadExc.dummyGlaSys.shade.tauSol_b"; zon1_roo_solRadExc_dummyG209 "zon1.roo.solRadExc.dummyGlaSys.shade.rhoSol_a"; zon1_roo_solRadExc_dummyG210 "zon1.roo.solRadExc.dummyGlaSys.shade.rhoSol_b"; zon1_roo_solRadExc_dummyG211 "zon1.roo.solRadExc.dummyGlaSys.shade.absIR_a"; zon1_roo_solRadExc_dummyG212 "zon1.roo.solRadExc.dummyGlaSys.shade.absIR_b"; zon1_roo_solRadExc_dummyG213 "zon1.roo.solRadExc.dummyGlaSys.shade.tauIR_a"; zon1_roo_solRadExc_dummyG214 "zon1.roo.solRadExc.dummyGlaSys.shade.tauIR_b"; zon1_roo_solRadExc_dummyG215 "zon1.roo.solRadExc.dummyGlaSys.UFra"; zon1_roo_solRadExc_dummyG216 "zon1.roo.solRadExc.dummyGlaSys.absIRFra"; zon1_roo_solRadExc_dummyG217 "zon1.roo.solRadExc.dummyGlaSys.absSolFra"; zon1_roo_irRadGai_datConE218 "zon1.roo.irRadGai.datConExtWin[1].ove.dep"; zon1_roo_irRadGai_datConE219 "zon1.roo.irRadGai.datConExtWin[1].sidFin.dep"; zon1_roo_irRadGai_dummyCo220 "zon1.roo.irRadGai.dummyCon.absIR_a"; zon1_roo_irRadGai_dummyCo221 "zon1.roo.irRadGai.dummyCon.absIR_b"; zon1_roo_irRadGai_dummyCo222 "zon1.roo.irRadGai.dummyCon.absSol_a"; zon1_roo_irRadGai_dummyCo223 "zon1.roo.irRadGai.dummyCon.absSol_b"; zon1_roo_irRadGai_dummyCo224 "zon1.roo.irRadGai.dummyCon.roughness_a"; zon1_roo_irRadGai_dummyGl225 "zon1.roo.irRadGai.dummyGlaSys.glass[1].x"; zon1_roo_irRadGai_dummyGl226 "zon1.roo.irRadGai.dummyGlaSys.glass[1].k"; zon1_roo_irRadGai_dummyGl227 "zon1.roo.irRadGai.dummyGlaSys.glass[1].tauSol"; zon1_roo_irRadGai_dummyGl228 "zon1.roo.irRadGai.dummyGlaSys.glass[1].rhoSol_a"; zon1_roo_irRadGai_dummyGl229 "zon1.roo.irRadGai.dummyGlaSys.glass[1].rhoSol_b"; zon1_roo_irRadGai_dummyGl230 "zon1.roo.irRadGai.dummyGlaSys.glass[1].tauIR"; zon1_roo_irRadGai_dummyGl231 "zon1.roo.irRadGai.dummyGlaSys.glass[1].absIR_a"; zon1_roo_irRadGai_dummyGl232 "zon1.roo.irRadGai.dummyGlaSys.glass[1].absIR_b"; zon1_roo_irRadGai_dummyGl233 "zon1.roo.irRadGai.dummyGlaSys.gas[1].x"; zon1_roo_irRadGai_dummyGl234 "zon1.roo.irRadGai.dummyGlaSys.gas[1].a_k"; zon1_roo_irRadGai_dummyGl235 "zon1.roo.irRadGai.dummyGlaSys.gas[1].b_k"; zon1_roo_irRadGai_dummyGl236 "zon1.roo.irRadGai.dummyGlaSys.gas[1].a_mu"; zon1_roo_irRadGai_dummyGl237 "zon1.roo.irRadGai.dummyGlaSys.gas[1].b_mu"; zon1_roo_irRadGai_dummyGl238 "zon1.roo.irRadGai.dummyGlaSys.gas[1].a_c"; zon1_roo_irRadGai_dummyGl239 "zon1.roo.irRadGai.dummyGlaSys.gas[1].b_c"; zon1_roo_irRadGai_dummyGl240 "zon1.roo.irRadGai.dummyGlaSys.gas[1].MM"; zon1_roo_irRadGai_dummyGl241 "zon1.roo.irRadGai.dummyGlaSys.gas[1].P0"; zon1_roo_irRadGai_dummyGl242 "zon1.roo.irRadGai.dummyGlaSys.shade.tauSol_a"; zon1_roo_irRadGai_dummyGl243 "zon1.roo.irRadGai.dummyGlaSys.shade.tauSol_b"; zon1_roo_irRadGai_dummyGl244 "zon1.roo.irRadGai.dummyGlaSys.shade.rhoSol_a"; zon1_roo_irRadGai_dummyGl245 "zon1.roo.irRadGai.dummyGlaSys.shade.rhoSol_b"; zon1_roo_irRadGai_dummyGl246 "zon1.roo.irRadGai.dummyGlaSys.shade.absIR_a"; zon1_roo_irRadGai_dummyGl247 "zon1.roo.irRadGai.dummyGlaSys.shade.absIR_b"; zon1_roo_irRadGai_dummyGl248 "zon1.roo.irRadGai.dummyGlaSys.shade.tauIR_a"; zon1_roo_irRadGai_dummyGl249 "zon1.roo.irRadGai.dummyGlaSys.shade.tauIR_b"; zon1_roo_irRadGai_dummyGl250 "zon1.roo.irRadGai.dummyGlaSys.UFra"; zon1_roo_irRadGai_dummyGl251 "zon1.roo.irRadGai.dummyGlaSys.absIRFra"; zon1_roo_irRadGai_dummyGl252 "zon1.roo.irRadGai.dummyGlaSys.absSolFra"; zon1_roo_irRadExc_datConE253 "zon1.roo.irRadExc.datConExtWin[1].ove.dep"; zon1_roo_irRadExc_datConE254 "zon1.roo.irRadExc.datConExtWin[1].sidFin.dep"; zon1_roo_irRadExc_dummyCo255 "zon1.roo.irRadExc.dummyCon.absIR_a"; zon1_roo_irRadExc_dummyCo256 "zon1.roo.irRadExc.dummyCon.absIR_b"; zon1_roo_irRadExc_dummyCo257 "zon1.roo.irRadExc.dummyCon.absSol_a"; zon1_roo_irRadExc_dummyCo258 "zon1.roo.irRadExc.dummyCon.absSol_b"; zon1_roo_irRadExc_dummyCo259 "zon1.roo.irRadExc.dummyCon.roughness_a"; zon1_roo_irRadExc_dummyGl260 "zon1.roo.irRadExc.dummyGlaSys.glass[1].x"; zon1_roo_irRadExc_dummyGl261 "zon1.roo.irRadExc.dummyGlaSys.glass[1].k"; zon1_roo_irRadExc_dummyGl262 "zon1.roo.irRadExc.dummyGlaSys.glass[1].tauSol"; zon1_roo_irRadExc_dummyGl263 "zon1.roo.irRadExc.dummyGlaSys.glass[1].rhoSol_a"; zon1_roo_irRadExc_dummyGl264 "zon1.roo.irRadExc.dummyGlaSys.glass[1].rhoSol_b"; zon1_roo_irRadExc_dummyGl265 "zon1.roo.irRadExc.dummyGlaSys.glass[1].tauIR"; zon1_roo_irRadExc_dummyGl266 "zon1.roo.irRadExc.dummyGlaSys.glass[1].absIR_a"; zon1_roo_irRadExc_dummyGl267 "zon1.roo.irRadExc.dummyGlaSys.glass[1].absIR_b"; zon1_roo_irRadExc_dummyGl268 "zon1.roo.irRadExc.dummyGlaSys.gas[1].x"; zon1_roo_irRadExc_dummyGl269 "zon1.roo.irRadExc.dummyGlaSys.gas[1].a_k"; zon1_roo_irRadExc_dummyGl270 "zon1.roo.irRadExc.dummyGlaSys.gas[1].b_k"; zon1_roo_irRadExc_dummyGl271 "zon1.roo.irRadExc.dummyGlaSys.gas[1].a_mu"; zon1_roo_irRadExc_dummyGl272 "zon1.roo.irRadExc.dummyGlaSys.gas[1].b_mu"; zon1_roo_irRadExc_dummyGl273 "zon1.roo.irRadExc.dummyGlaSys.gas[1].a_c"; zon1_roo_irRadExc_dummyGl274 "zon1.roo.irRadExc.dummyGlaSys.gas[1].b_c"; zon1_roo_irRadExc_dummyGl275 "zon1.roo.irRadExc.dummyGlaSys.gas[1].MM"; zon1_roo_irRadExc_dummyGl276 "zon1.roo.irRadExc.dummyGlaSys.gas[1].P0"; zon1_roo_irRadExc_dummyGl277 "zon1.roo.irRadExc.dummyGlaSys.shade.tauSol_a"; zon1_roo_irRadExc_dummyGl278 "zon1.roo.irRadExc.dummyGlaSys.shade.tauSol_b"; zon1_roo_irRadExc_dummyGl279 "zon1.roo.irRadExc.dummyGlaSys.shade.rhoSol_a"; zon1_roo_irRadExc_dummyGl280 "zon1.roo.irRadExc.dummyGlaSys.shade.rhoSol_b"; zon1_roo_irRadExc_dummyGl281 "zon1.roo.irRadExc.dummyGlaSys.shade.absIR_a"; zon1_roo_irRadExc_dummyGl282 "zon1.roo.irRadExc.dummyGlaSys.shade.absIR_b"; zon1_roo_irRadExc_dummyGl283 "zon1.roo.irRadExc.dummyGlaSys.shade.tauIR_a"; zon1_roo_irRadExc_dummyGl284 "zon1.roo.irRadExc.dummyGlaSys.shade.tauIR_b"; zon1_roo_irRadExc_dummyGl285 "zon1.roo.irRadExc.dummyGlaSys.UFra"; zon1_roo_irRadExc_dummyGl286 "zon1.roo.irRadExc.dummyGlaSys.absIRFra"; zon1_roo_irRadExc_dummyGl287 "zon1.roo.irRadExc.dummyGlaSys.absSolFra"; zon1_roo_irRadExc_T0 "zon1.roo.irRadExc.T0"; zon1_roo_radTem_datConExt289 "zon1.roo.radTem.datConExtWin[1].ove.dep"; zon1_roo_radTem_datConExt290 "zon1.roo.radTem.datConExtWin[1].sidFin.dep"; zon1_roo_radTem_dummyCon_291 "zon1.roo.radTem.dummyCon.absIR_a"; zon1_roo_radTem_dummyCon_292 "zon1.roo.radTem.dummyCon.absIR_b"; zon1_roo_radTem_dummyCon_293 "zon1.roo.radTem.dummyCon.absSol_a"; zon1_roo_radTem_dummyCon_294 "zon1.roo.radTem.dummyCon.absSol_b"; zon1_roo_radTem_dummyCon_295 "zon1.roo.radTem.dummyCon.roughness_a"; zon1_roo_radTem_dummyGlaS296 "zon1.roo.radTem.dummyGlaSys.glass[1].x"; zon1_roo_radTem_dummyGlaS297 "zon1.roo.radTem.dummyGlaSys.glass[1].k"; zon1_roo_radTem_dummyGlaS298 "zon1.roo.radTem.dummyGlaSys.glass[1].tauSol"; zon1_roo_radTem_dummyGlaS299 "zon1.roo.radTem.dummyGlaSys.glass[1].rhoSol_a"; zon1_roo_radTem_dummyGlaS300 "zon1.roo.radTem.dummyGlaSys.glass[1].rhoSol_b"; zon1_roo_radTem_dummyGlaS301 "zon1.roo.radTem.dummyGlaSys.glass[1].tauIR"; zon1_roo_radTem_dummyGlaS302 "zon1.roo.radTem.dummyGlaSys.glass[1].absIR_a"; zon1_roo_radTem_dummyGlaS303 "zon1.roo.radTem.dummyGlaSys.glass[1].absIR_b"; zon1_roo_radTem_dummyGlaS304 "zon1.roo.radTem.dummyGlaSys.gas[1].x"; zon1_roo_radTem_dummyGlaS305 "zon1.roo.radTem.dummyGlaSys.gas[1].a_k"; zon1_roo_radTem_dummyGlaS306 "zon1.roo.radTem.dummyGlaSys.gas[1].b_k"; zon1_roo_radTem_dummyGlaS307 "zon1.roo.radTem.dummyGlaSys.gas[1].a_mu"; zon1_roo_radTem_dummyGlaS308 "zon1.roo.radTem.dummyGlaSys.gas[1].b_mu"; zon1_roo_radTem_dummyGlaS309 "zon1.roo.radTem.dummyGlaSys.gas[1].a_c"; zon1_roo_radTem_dummyGlaS310 "zon1.roo.radTem.dummyGlaSys.gas[1].b_c"; zon1_roo_radTem_dummyGlaS311 "zon1.roo.radTem.dummyGlaSys.gas[1].MM"; zon1_roo_radTem_dummyGlaS312 "zon1.roo.radTem.dummyGlaSys.gas[1].P0"; zon1_roo_radTem_dummyGlaS313 "zon1.roo.radTem.dummyGlaSys.shade.tauSol_a"; zon1_roo_radTem_dummyGlaS314 "zon1.roo.radTem.dummyGlaSys.shade.tauSol_b"; zon1_roo_radTem_dummyGlaS315 "zon1.roo.radTem.dummyGlaSys.shade.rhoSol_a"; zon1_roo_radTem_dummyGlaS316 "zon1.roo.radTem.dummyGlaSys.shade.rhoSol_b"; zon1_roo_radTem_dummyGlaS317 "zon1.roo.radTem.dummyGlaSys.shade.absIR_a"; zon1_roo_radTem_dummyGlaS318 "zon1.roo.radTem.dummyGlaSys.shade.absIR_b"; zon1_roo_radTem_dummyGlaS319 "zon1.roo.radTem.dummyGlaSys.shade.tauIR_a"; zon1_roo_radTem_dummyGlaS320 "zon1.roo.radTem.dummyGlaSys.shade.tauIR_b"; zon1_roo_radTem_dummyGlaS321 "zon1.roo.radTem.dummyGlaSys.UFra"; zon1_roo_radTem_dummyGlaS322 "zon1.roo.radTem.dummyGlaSys.absIRFra"; zon1_roo_radTem_dummyGlaS323 "zon1.roo.radTem.dummyGlaSys.absSolFra"; zon1_roo_add_k1 "zon1.roo.add.k1"; zon1_roo_add_k2 "zon1.roo.add.k2"; zon1_roo_sumJFroWin_1__k "zon1.roo.sumJFroWin[1].k"; zon1_roo_p_start "zon1.roo.p_start"; zon1_roo_T_start "zon1.roo.T_start"; zon1_roo_X_start "zon1.roo.X_start"; zon1_qConGai_flow_k "zon1.qConGai_flow.k"; zon1_qRadGai_flow_k "zon1.qRadGai_flow.k"; zon1_qLatGai_flow_k "zon1.qLatGai_flow.k"; zon1_TSoi_1__T "zon1.TSoi[1].T"; zon1_sinInf_m_flow "zon1.sinInf.m_flow"; zon1_sinInf_x_pTphi_p "zon1.sinInf.x_pTphi.p"; zon1_InfiltrationRate_k "zon1.InfiltrationRate.k"; zon1_souInf_m_flow "zon1.souInf.m_flow"; zon1_souInf_x_pTphi_p "zon1.souInf.x_pTphi.p"; zon1_intLoad_table "zon1.intLoad.table"; zon1_intLoad_verboseRead "zon1.intLoad.verboseRead"; zon1_intLoad_columns "zon1.intLoad.columns"; zon1_intLoad_offset "zon1.intLoad.offset"; zon1_intLoad_startTime "zon1.intLoad.startTime"; zon1_intLoad_timeEvents "zon1.intLoad.timeEvents"; coiSou_X "coiSou.X"; coiSou_T "coiSou.T"; res_sta_default_p "res.sta_default.p"; res_sta_default_T "res.sta_default.T"; res_sta_default_X "res.sta_default.X"; weaDat_lon "weaDat.lon"; weaDat_lat "weaDat.lat"; weaDat_wea_table "weaDat.wea.table"; weaDat_wea_verboseRead "weaDat.wea.verboseRead"; weaDat_wea_offset "weaDat.wea.offset"; weaDat_wea_startTime "weaDat.wea.startTime"; weaDat_wea_timeEvents "weaDat.wea.timeEvents"; sin_X "sin.X"; sin_p "sin.p"; sin_T "sin.T"; vav1_vav_sta_default_p "vav1.vav.sta_default.p"; vav1_vav_sta_default_T "vav1.vav.sta_default.T"; vav1_vav_sta_default_X "vav1.vav.sta_default.X"; vav1_vav_riseTime "vav1.vav.riseTime"; vav1_vav_y_start "vav1.vav.y_start"; vav1_vav_filter_gain "vav1.vav.filter.gain"; vav1_vav_filter_A_ripple "vav1.vav.filter.A_ripple"; vav1_vav_filter_f_min "vav1.vav.filter.f_min"; vav1_vav_filter_normalize368 "vav1.vav.filter.normalized"; vav1_vav_filter_x_start "vav1.vav.filter.x_start"; vav1_vav_filter_u_nominal "vav1.vav.filter.u_nominal"; vav1_vav_use_deltaM "vav1.vav.use_deltaM"; vav1_vav_deltaM "vav1.vav.deltaM"; vav1_vav_roundDuct "vav1.vav.roundDuct"; vav1_vav_ReC "vav1.vav.ReC"; vav1_vav_a "vav1.vav.a"; vav1_vav_b "vav1.vav.b"; vav1_vav_yL "vav1.vav.yL"; vav1_vav_yU "vav1.vav.yU"; vav1_vav_k1 "vav1.vav.k1"; vav1_vav_l "vav1.vav.l"; vav1_vav_l2 "vav1.vav.l2"; vav1_vav_deltax "vav1.vav.deltax"; vav1_vav_y_min "vav1.vav.y_min"; vav1_terHea_bal1_preDro_s384 "vav1.terHea.bal1.preDro.sta_default.p"; vav1_terHea_bal1_preDro_s385 "vav1.terHea.bal1.preDro.sta_default.T"; vav1_terHea_bal1_preDro_s386 "vav1.terHea.bal1.preDro.sta_default.X"; vav1_terHea_bal2_preDro_s387 "vav1.terHea.bal2.preDro.sta_default.p"; vav1_terHea_bal2_preDro_s388 "vav1.terHea.bal2.preDro.sta_default.T"; vav1_terHea_delta "vav1.terHea.delta"; vav1_terHea_T_a1_nominal "vav1.terHea.T_a1_nominal"; vav1_terHea_T_a2_nominal "vav1.terHea.T_a2_nominal"; vav1_terHea_r_nominal "vav1.terHea.r_nominal"; vav1_terHea_hA_n_w "vav1.terHea.hA.n_w"; vav1_terHea_hA_n_a "vav1.terHea.hA.n_a"; vav1_terHea_hA_T0_w "vav1.terHea.hA.T0_w"; vav1_terHea_hA_T0_a "vav1.terHea.hA.T0_a"; vav1_sinTer_X "vav1.sinTer.X"; vav1_sinTer_p "vav1.sinTer.p"; vav1_sinTer_T "vav1.sinTer.T"; vav1_souTer_X "vav1.souTer.X"; vav1_souTer_m_flow "vav1.souTer.m_flow"; vav1_souTer_T "vav1.souTer.T"; VSup1_T_start "VSup1.T_start"; VSup1_p_start "VSup1.p_start"; VSup1_X_start "VSup1.X_start"; TDisVAV1_T_start "TDisVAV1.T_start"; TDisVAV1_TAmb "TDisVAV1.TAmb"; TDisVAV1_tauHeaTra "TDisVAV1.tauHeaTra"; zer_k "zer.k"; vav2_vav_sta_default_p "vav2.vav.sta_default.p"; vav2_vav_sta_default_T "vav2.vav.sta_default.T"; vav2_vav_sta_default_X "vav2.vav.sta_default.X"; vav2_vav_riseTime "vav2.vav.riseTime"; vav2_vav_y_start "vav2.vav.y_start"; vav2_vav_filter_gain "vav2.vav.filter.gain"; vav2_vav_filter_A_ripple "vav2.vav.filter.A_ripple"; vav2_vav_filter_f_min "vav2.vav.filter.f_min"; vav2_vav_filter_normalize418 "vav2.vav.filter.normalized"; vav2_vav_filter_x_start "vav2.vav.filter.x_start"; vav2_vav_filter_u_nominal "vav2.vav.filter.u_nominal"; vav2_vav_use_deltaM "vav2.vav.use_deltaM"; vav2_vav_deltaM "vav2.vav.deltaM"; vav2_vav_roundDuct "vav2.vav.roundDuct"; vav2_vav_ReC "vav2.vav.ReC"; vav2_vav_a "vav2.vav.a"; vav2_vav_b "vav2.vav.b"; vav2_vav_yL "vav2.vav.yL"; vav2_vav_yU "vav2.vav.yU"; vav2_vav_k1 "vav2.vav.k1"; vav2_vav_l "vav2.vav.l"; vav2_vav_l2 "vav2.vav.l2"; vav2_vav_deltax "vav2.vav.deltax"; vav2_vav_y_min "vav2.vav.y_min"; vav2_terHea_bal1_preDro_s434 "vav2.terHea.bal1.preDro.sta_default.p"; vav2_terHea_bal1_preDro_s435 "vav2.terHea.bal1.preDro.sta_default.T"; vav2_terHea_bal1_preDro_s436 "vav2.terHea.bal1.preDro.sta_default.X"; vav2_terHea_bal2_preDro_s437 "vav2.terHea.bal2.preDro.sta_default.p"; vav2_terHea_bal2_preDro_s438 "vav2.terHea.bal2.preDro.sta_default.T"; vav2_terHea_delta "vav2.terHea.delta"; vav2_terHea_T_a1_nominal "vav2.terHea.T_a1_nominal"; vav2_terHea_T_a2_nominal "vav2.terHea.T_a2_nominal"; vav2_terHea_r_nominal "vav2.terHea.r_nominal"; vav2_terHea_hA_n_w "vav2.terHea.hA.n_w"; vav2_terHea_hA_n_a "vav2.terHea.hA.n_a"; vav2_terHea_hA_T0_w "vav2.terHea.hA.T0_w"; vav2_terHea_hA_T0_a "vav2.terHea.hA.T0_a"; vav2_sinTer_X "vav2.sinTer.X"; vav2_sinTer_p "vav2.sinTer.p"; vav2_sinTer_T "vav2.sinTer.T"; vav2_souTer_X "vav2.souTer.X"; vav2_souTer_m_flow "vav2.souTer.m_flow"; vav2_souTer_T "vav2.souTer.T"; TDisVAV2_T_start "TDisVAV2.T_start"; TDisVAV2_TAmb "TDisVAV2.TAmb"; TDisVAV2_tauHeaTra "TDisVAV2.tauHeaTra"; VSup2_T_start "VSup2.T_start"; VSup2_p_start "VSup2.p_start"; VSup2_X_start "VSup2.X_start"; zon2_S_ "zon2.S_"; zon2_E_ "zon2.E_"; zon2_W_ "zon2.W_"; zon2_N_ "zon2.N_"; zon2_matExtWal_absIR_a "zon2.matExtWal.absIR_a"; zon2_matExtWal_absIR_b "zon2.matExtWal.absIR_b"; zon2_matExtWal_absSol_a "zon2.matExtWal.absSol_a"; zon2_matExtWal_absSol_b "zon2.matExtWal.absSol_b"; zon2_matExtWal_roughness_467 "zon2.matExtWal.roughness_a"; zon2_matFlo_absIR_a "zon2.matFlo.absIR_a"; zon2_matFlo_absIR_b "zon2.matFlo.absIR_b"; zon2_matFlo_absSol_a "zon2.matFlo.absSol_a"; zon2_matFlo_absSol_b "zon2.matFlo.absSol_b"; zon2_matFlo_roughness_a "zon2.matFlo.roughness_a"; zon2_roof_absIR_a "zon2.roof.absIR_a"; zon2_roof_absIR_b "zon2.roof.absIR_b"; zon2_roof_absSol_a "zon2.roof.absSol_a"; zon2_roof_absSol_b "zon2.roof.absSol_b"; zon2_roof_roughness_a "zon2.roof.roughness_a"; zon2_window600_glass_1__x "zon2.window600.glass[1].x"; zon2_window600_glass_1__k "zon2.window600.glass[1].k"; zon2_window600_glass_1__t480 "zon2.window600.glass[1].tauSol"; zon2_window600_glass_1__r481 "zon2.window600.glass[1].rhoSol_a"; zon2_window600_glass_1__r482 "zon2.window600.glass[1].rhoSol_b"; zon2_window600_glass_1__t483 "zon2.window600.glass[1].tauIR"; zon2_window600_glass_1__a484 "zon2.window600.glass[1].absIR_a"; zon2_window600_glass_1__a485 "zon2.window600.glass[1].absIR_b"; zon2_window600_glass_2__x "zon2.window600.glass[2].x"; zon2_window600_glass_2__k "zon2.window600.glass[2].k"; zon2_window600_glass_2__t488 "zon2.window600.glass[2].tauSol"; zon2_window600_glass_2__r489 "zon2.window600.glass[2].rhoSol_a"; zon2_window600_glass_2__r490 "zon2.window600.glass[2].rhoSol_b"; zon2_window600_glass_2__t491 "zon2.window600.glass[2].tauIR"; zon2_window600_glass_2__a492 "zon2.window600.glass[2].absIR_a"; zon2_window600_glass_2__a493 "zon2.window600.glass[2].absIR_b"; zon2_window600_gas_1__x "zon2.window600.gas[1].x"; zon2_window600_gas_1__a_k "zon2.window600.gas[1].a_k"; zon2_window600_gas_1__b_k "zon2.window600.gas[1].b_k"; zon2_window600_gas_1__a_m497 "zon2.window600.gas[1].a_mu"; zon2_window600_gas_1__b_m498 "zon2.window600.gas[1].b_mu"; zon2_window600_gas_1__a_c "zon2.window600.gas[1].a_c"; zon2_window600_gas_1__b_c "zon2.window600.gas[1].b_c"; zon2_window600_gas_1__MM "zon2.window600.gas[1].MM"; zon2_window600_gas_1__P0 "zon2.window600.gas[1].P0"; zon2_window600_shade_tauS503 "zon2.window600.shade.tauSol_a"; zon2_window600_shade_tauS504 "zon2.window600.shade.tauSol_b"; zon2_window600_shade_rhoS505 "zon2.window600.shade.rhoSol_a"; zon2_window600_shade_rhoS506 "zon2.window600.shade.rhoSol_b"; zon2_window600_shade_absI507 "zon2.window600.shade.absIR_a"; zon2_window600_shade_absI508 "zon2.window600.shade.absIR_b"; zon2_window600_shade_tauI509 "zon2.window600.shade.tauIR_a"; zon2_window600_shade_tauI510 "zon2.window600.shade.tauIR_b"; zon2_window600_UFra "zon2.window600.UFra"; zon2_window600_absIRFra "zon2.window600.absIRFra"; zon2_window600_absSolFra "zon2.window600.absSolFra"; zon2_soi_A "zon2.soi.A"; zon2_soi_T_a_start "zon2.soi.T_a_start"; zon2_soi_T_b_start "zon2.soi.T_b_start"; zon2_roo_datConExt_1__bou517 "zon2.roo.datConExt[1].boundaryCondition"; zon2_roo_datConExt_1__A "zon2.roo.datConExt[1].A"; zon2_roo_datConExt_2__bou519 "zon2.roo.datConExt[2].boundaryCondition"; zon2_roo_datConExt_2__A "zon2.roo.datConExt[2].A"; zon2_roo_datConExt_3__bou521 "zon2.roo.datConExt[3].boundaryCondition"; zon2_roo_datConExt_3__A "zon2.roo.datConExt[3].A"; zon2_roo_datConExt_4__bou523 "zon2.roo.datConExt[4].boundaryCondition"; zon2_roo_datConExt_4__A "zon2.roo.datConExt[4].A"; zon2_roo_datConExtWin_1__525 "zon2.roo.datConExtWin[1].boundaryCondition"; zon2_roo_datConExtWin_1__526 "zon2.roo.datConExtWin[1].A"; zon2_roo_datConExtWin_1__527 "zon2.roo.datConExtWin[1].hWin"; zon2_roo_datConExtWin_1__528 "zon2.roo.datConExtWin[1].wWin"; zon2_roo_datConExtWin_1__529 "zon2.roo.datConExtWin[1].fFra"; zon2_roo_datConExtWin_1__530 "zon2.roo.datConExtWin[1].ove.wL"; zon2_roo_datConExtWin_1__531 "zon2.roo.datConExtWin[1].ove.wR"; zon2_roo_datConExtWin_1__532 "zon2.roo.datConExtWin[1].ove.gap"; zon2_roo_datConExtWin_1__533 "zon2.roo.datConExtWin[1].sidFin.h"; zon2_roo_datConExtWin_1__534 "zon2.roo.datConExtWin[1].sidFin.gap"; zon2_roo_datConPar_1__azi "zon2.roo.datConPar[1].azi"; zon2_roo_datConPar_1__bou536 "zon2.roo.datConPar[1].boundaryCondition"; zon2_roo_datConPar_1__A "zon2.roo.datConPar[1].A"; zon2_roo_datConBou_1__azi "zon2.roo.datConBou[1].azi"; zon2_roo_datConBou_1__bou539 "zon2.roo.datConBou[1].boundaryCondition"; zon2_roo_datConBou_1__A "zon2.roo.datConBou[1].A"; zon2_roo_surBou_1__A "zon2.roo.surBou[1].A"; zon2_roo_surBou_1__absIR "zon2.roo.surBou[1].absIR"; zon2_roo_surBou_1__absSol "zon2.roo.surBou[1].absSol"; zon2_roo_surBou_1__bounda544 "zon2.roo.surBou[1].boundaryCondition"; zon2_roo_dummyCon_absIR_a "zon2.roo.dummyCon.absIR_a"; zon2_roo_dummyCon_absIR_b "zon2.roo.dummyCon.absIR_b"; zon2_roo_dummyCon_absSol_547 "zon2.roo.dummyCon.absSol_a"; zon2_roo_dummyCon_absSol_548 "zon2.roo.dummyCon.absSol_b"; zon2_roo_dummyCon_roughne549 "zon2.roo.dummyCon.roughness_a"; zon2_roo_dummyGlaSys_glas550 "zon2.roo.dummyGlaSys.glass[1].x"; zon2_roo_dummyGlaSys_glas551 "zon2.roo.dummyGlaSys.glass[1].k"; zon2_roo_dummyGlaSys_glas552 "zon2.roo.dummyGlaSys.glass[1].tauSol"; zon2_roo_dummyGlaSys_glas553 "zon2.roo.dummyGlaSys.glass[1].rhoSol_a"; zon2_roo_dummyGlaSys_glas554 "zon2.roo.dummyGlaSys.glass[1].rhoSol_b"; zon2_roo_dummyGlaSys_glas555 "zon2.roo.dummyGlaSys.glass[1].tauIR"; zon2_roo_dummyGlaSys_glas556 "zon2.roo.dummyGlaSys.glass[1].absIR_a"; zon2_roo_dummyGlaSys_glas557 "zon2.roo.dummyGlaSys.glass[1].absIR_b"; zon2_roo_dummyGlaSys_gas_558 "zon2.roo.dummyGlaSys.gas[1].x"; zon2_roo_dummyGlaSys_gas_559 "zon2.roo.dummyGlaSys.gas[1].a_k"; zon2_roo_dummyGlaSys_gas_560 "zon2.roo.dummyGlaSys.gas[1].b_k"; zon2_roo_dummyGlaSys_gas_561 "zon2.roo.dummyGlaSys.gas[1].a_mu"; zon2_roo_dummyGlaSys_gas_562 "zon2.roo.dummyGlaSys.gas[1].b_mu"; zon2_roo_dummyGlaSys_gas_563 "zon2.roo.dummyGlaSys.gas[1].a_c"; zon2_roo_dummyGlaSys_gas_564 "zon2.roo.dummyGlaSys.gas[1].b_c"; zon2_roo_dummyGlaSys_gas_565 "zon2.roo.dummyGlaSys.gas[1].MM"; zon2_roo_dummyGlaSys_gas_566 "zon2.roo.dummyGlaSys.gas[1].P0"; zon2_roo_dummyGlaSys_shad567 "zon2.roo.dummyGlaSys.shade.tauSol_a"; zon2_roo_dummyGlaSys_shad568 "zon2.roo.dummyGlaSys.shade.tauSol_b"; zon2_roo_dummyGlaSys_shad569 "zon2.roo.dummyGlaSys.shade.rhoSol_a"; zon2_roo_dummyGlaSys_shad570 "zon2.roo.dummyGlaSys.shade.rhoSol_b"; zon2_roo_dummyGlaSys_shad571 "zon2.roo.dummyGlaSys.shade.absIR_a"; zon2_roo_dummyGlaSys_shad572 "zon2.roo.dummyGlaSys.shade.absIR_b"; zon2_roo_dummyGlaSys_shad573 "zon2.roo.dummyGlaSys.shade.tauIR_a"; zon2_roo_dummyGlaSys_shad574 "zon2.roo.dummyGlaSys.shade.tauIR_b"; zon2_roo_dummyGlaSys_UFra "zon2.roo.dummyGlaSys.UFra"; zon2_roo_dummyGlaSys_absI576 "zon2.roo.dummyGlaSys.absIRFra"; zon2_roo_dummyGlaSys_absS577 "zon2.roo.dummyGlaSys.absSolFra"; zon2_roo_AFlo "zon2.roo.AFlo"; zon2_roo_hRoo "zon2.roo.hRoo"; zon2_roo_conExtWin_1__gla580 "zon2.roo.conExtWin[1].glaSys.haveControllableWindow"; zon2_roo_conExtWin_1__win581 "zon2.roo.conExtWin[1].win.matGla.k"; zon2_roo_conExtWin_1__win582 "zon2.roo.conExtWin[1].win.matGla.nStaRef"; zon2_roo_conExtWin_1__win583 "zon2.roo.conExtWin[1].win.matGla.piRef"; zon2_roo_conExtWin_1__win584 "zon2.roo.conExtWin[1].win.matGla.nStaReal"; zon2_roo_hIntFixed "zon2.roo.hIntFixed"; zon2_roo_hExtFixed "zon2.roo.hExtFixed"; zon2_roo_bouConExt_HDifTi587 "zon2.roo.bouConExt.HDifTil[1].rho"; zon2_roo_bouConExt_HDifTi588 "zon2.roo.bouConExt.HDifTil[1].add.k1"; zon2_roo_bouConExt_HDifTi589 "zon2.roo.bouConExt.HDifTil[1].add.k2"; zon2_roo_bouConExt_HDifTi590 "zon2.roo.bouConExt.HDifTil[2].rho"; zon2_roo_bouConExt_HDifTi591 "zon2.roo.bouConExt.HDifTil[2].add.k1"; zon2_roo_bouConExt_HDifTi592 "zon2.roo.bouConExt.HDifTil[2].add.k2"; zon2_roo_bouConExt_HDifTi593 "zon2.roo.bouConExt.HDifTil[3].rho"; zon2_roo_bouConExt_HDifTi594 "zon2.roo.bouConExt.HDifTil[3].add.k1"; zon2_roo_bouConExt_HDifTi595 "zon2.roo.bouConExt.HDifTil[3].add.k2"; zon2_roo_bouConExt_HDifTi596 "zon2.roo.bouConExt.HDifTil[4].rho"; zon2_roo_bouConExt_HDifTi597 "zon2.roo.bouConExt.HDifTil[4].add.k1"; zon2_roo_bouConExt_HDifTi598 "zon2.roo.bouConExt.HDifTil[4].add.k2"; zon2_roo_bouConExtWin_con599 "zon2.roo.bouConExtWin.conPar[1].ove.dep"; zon2_roo_bouConExtWin_con600 "zon2.roo.bouConExtWin.conPar[1].sidFin.dep"; zon2_roo_bouConExtWin_HDi601 "zon2.roo.bouConExtWin.HDifTil[1].rho"; zon2_roo_bouConExtWin_HDi602 "zon2.roo.bouConExtWin.HDifTil[1].add.k1"; zon2_roo_bouConExtWin_HDi603 "zon2.roo.bouConExtWin.HDifTil[1].add.k2"; zon2_roo_bouConExtWin_con604 "zon2.roo.bouConExtWin.conExtWin[1].radOut.T0"; zon2_roo_air_datConExtWin605 "zon2.roo.air.datConExtWin[1].ove.dep"; zon2_roo_air_datConExtWin606 "zon2.roo.air.datConExtWin[1].sidFin.dep"; zon2_roo_air_dummyCon_abs607 "zon2.roo.air.dummyCon.absIR_a"; zon2_roo_air_dummyCon_abs608 "zon2.roo.air.dummyCon.absIR_b"; zon2_roo_air_dummyCon_abs609 "zon2.roo.air.dummyCon.absSol_a"; zon2_roo_air_dummyCon_abs610 "zon2.roo.air.dummyCon.absSol_b"; zon2_roo_air_dummyCon_rou611 "zon2.roo.air.dummyCon.roughness_a"; zon2_roo_air_dummyGlaSys_612 "zon2.roo.air.dummyGlaSys.glass[1].x"; zon2_roo_air_dummyGlaSys_613 "zon2.roo.air.dummyGlaSys.glass[1].k"; zon2_roo_air_dummyGlaSys_614 "zon2.roo.air.dummyGlaSys.glass[1].tauSol"; zon2_roo_air_dummyGlaSys_615 "zon2.roo.air.dummyGlaSys.glass[1].rhoSol_a"; zon2_roo_air_dummyGlaSys_616 "zon2.roo.air.dummyGlaSys.glass[1].rhoSol_b"; zon2_roo_air_dummyGlaSys_617 "zon2.roo.air.dummyGlaSys.glass[1].tauIR"; zon2_roo_air_dummyGlaSys_618 "zon2.roo.air.dummyGlaSys.glass[1].absIR_a"; zon2_roo_air_dummyGlaSys_619 "zon2.roo.air.dummyGlaSys.glass[1].absIR_b"; zon2_roo_air_dummyGlaSys_620 "zon2.roo.air.dummyGlaSys.gas[1].x"; zon2_roo_air_dummyGlaSys_621 "zon2.roo.air.dummyGlaSys.gas[1].a_k"; zon2_roo_air_dummyGlaSys_622 "zon2.roo.air.dummyGlaSys.gas[1].b_k"; zon2_roo_air_dummyGlaSys_623 "zon2.roo.air.dummyGlaSys.gas[1].a_mu"; zon2_roo_air_dummyGlaSys_624 "zon2.roo.air.dummyGlaSys.gas[1].b_mu"; zon2_roo_air_dummyGlaSys_625 "zon2.roo.air.dummyGlaSys.gas[1].a_c"; zon2_roo_air_dummyGlaSys_626 "zon2.roo.air.dummyGlaSys.gas[1].b_c"; zon2_roo_air_dummyGlaSys_627 "zon2.roo.air.dummyGlaSys.gas[1].MM"; zon2_roo_air_dummyGlaSys_628 "zon2.roo.air.dummyGlaSys.gas[1].P0"; zon2_roo_air_dummyGlaSys_629 "zon2.roo.air.dummyGlaSys.shade.tauSol_a"; zon2_roo_air_dummyGlaSys_630 "zon2.roo.air.dummyGlaSys.shade.tauSol_b"; zon2_roo_air_dummyGlaSys_631 "zon2.roo.air.dummyGlaSys.shade.rhoSol_a"; zon2_roo_air_dummyGlaSys_632 "zon2.roo.air.dummyGlaSys.shade.rhoSol_b"; zon2_roo_air_dummyGlaSys_633 "zon2.roo.air.dummyGlaSys.shade.absIR_a"; zon2_roo_air_dummyGlaSys_634 "zon2.roo.air.dummyGlaSys.shade.absIR_b"; zon2_roo_air_dummyGlaSys_635 "zon2.roo.air.dummyGlaSys.shade.tauIR_a"; zon2_roo_air_dummyGlaSys_636 "zon2.roo.air.dummyGlaSys.shade.tauIR_b"; zon2_roo_air_dummyGlaSys_637 "zon2.roo.air.dummyGlaSys.UFra"; zon2_roo_air_dummyGlaSys_638 "zon2.roo.air.dummyGlaSys.absIRFra"; zon2_roo_air_dummyGlaSys_639 "zon2.roo.air.dummyGlaSys.absSolFra"; zon2_roo_solRadExc_datCon640 "zon2.roo.solRadExc.datConExtWin[1].ove.dep"; zon2_roo_solRadExc_datCon641 "zon2.roo.solRadExc.datConExtWin[1].sidFin.dep"; zon2_roo_solRadExc_dummyC642 "zon2.roo.solRadExc.dummyCon.absIR_a"; zon2_roo_solRadExc_dummyC643 "zon2.roo.solRadExc.dummyCon.absIR_b"; zon2_roo_solRadExc_dummyC644 "zon2.roo.solRadExc.dummyCon.absSol_a"; zon2_roo_solRadExc_dummyC645 "zon2.roo.solRadExc.dummyCon.absSol_b"; zon2_roo_solRadExc_dummyC646 "zon2.roo.solRadExc.dummyCon.roughness_a"; zon2_roo_solRadExc_dummyG647 "zon2.roo.solRadExc.dummyGlaSys.glass[1].x"; zon2_roo_solRadExc_dummyG648 "zon2.roo.solRadExc.dummyGlaSys.glass[1].k"; zon2_roo_solRadExc_dummyG649 "zon2.roo.solRadExc.dummyGlaSys.glass[1].tauSol"; zon2_roo_solRadExc_dummyG650 "zon2.roo.solRadExc.dummyGlaSys.glass[1].rhoSol_a"; zon2_roo_solRadExc_dummyG651 "zon2.roo.solRadExc.dummyGlaSys.glass[1].rhoSol_b"; zon2_roo_solRadExc_dummyG652 "zon2.roo.solRadExc.dummyGlaSys.glass[1].tauIR"; zon2_roo_solRadExc_dummyG653 "zon2.roo.solRadExc.dummyGlaSys.glass[1].absIR_a"; zon2_roo_solRadExc_dummyG654 "zon2.roo.solRadExc.dummyGlaSys.glass[1].absIR_b"; zon2_roo_solRadExc_dummyG655 "zon2.roo.solRadExc.dummyGlaSys.gas[1].x"; zon2_roo_solRadExc_dummyG656 "zon2.roo.solRadExc.dummyGlaSys.gas[1].a_k"; zon2_roo_solRadExc_dummyG657 "zon2.roo.solRadExc.dummyGlaSys.gas[1].b_k"; zon2_roo_solRadExc_dummyG658 "zon2.roo.solRadExc.dummyGlaSys.gas[1].a_mu"; zon2_roo_solRadExc_dummyG659 "zon2.roo.solRadExc.dummyGlaSys.gas[1].b_mu"; zon2_roo_solRadExc_dummyG660 "zon2.roo.solRadExc.dummyGlaSys.gas[1].a_c"; zon2_roo_solRadExc_dummyG661 "zon2.roo.solRadExc.dummyGlaSys.gas[1].b_c"; zon2_roo_solRadExc_dummyG662 "zon2.roo.solRadExc.dummyGlaSys.gas[1].MM"; zon2_roo_solRadExc_dummyG663 "zon2.roo.solRadExc.dummyGlaSys.gas[1].P0"; zon2_roo_solRadExc_dummyG664 "zon2.roo.solRadExc.dummyGlaSys.shade.tauSol_a"; zon2_roo_solRadExc_dummyG665 "zon2.roo.solRadExc.dummyGlaSys.shade.tauSol_b"; zon2_roo_solRadExc_dummyG666 "zon2.roo.solRadExc.dummyGlaSys.shade.rhoSol_a"; zon2_roo_solRadExc_dummyG667 "zon2.roo.solRadExc.dummyGlaSys.shade.rhoSol_b"; zon2_roo_solRadExc_dummyG668 "zon2.roo.solRadExc.dummyGlaSys.shade.absIR_a"; zon2_roo_solRadExc_dummyG669 "zon2.roo.solRadExc.dummyGlaSys.shade.absIR_b"; zon2_roo_solRadExc_dummyG670 "zon2.roo.solRadExc.dummyGlaSys.shade.tauIR_a"; zon2_roo_solRadExc_dummyG671 "zon2.roo.solRadExc.dummyGlaSys.shade.tauIR_b"; zon2_roo_solRadExc_dummyG672 "zon2.roo.solRadExc.dummyGlaSys.UFra"; zon2_roo_solRadExc_dummyG673 "zon2.roo.solRadExc.dummyGlaSys.absIRFra"; zon2_roo_solRadExc_dummyG674 "zon2.roo.solRadExc.dummyGlaSys.absSolFra"; zon2_roo_irRadGai_datConE675 "zon2.roo.irRadGai.datConExtWin[1].ove.dep"; zon2_roo_irRadGai_datConE676 "zon2.roo.irRadGai.datConExtWin[1].sidFin.dep"; zon2_roo_irRadGai_dummyCo677 "zon2.roo.irRadGai.dummyCon.absIR_a"; zon2_roo_irRadGai_dummyCo678 "zon2.roo.irRadGai.dummyCon.absIR_b"; zon2_roo_irRadGai_dummyCo679 "zon2.roo.irRadGai.dummyCon.absSol_a"; zon2_roo_irRadGai_dummyCo680 "zon2.roo.irRadGai.dummyCon.absSol_b"; zon2_roo_irRadGai_dummyCo681 "zon2.roo.irRadGai.dummyCon.roughness_a"; zon2_roo_irRadGai_dummyGl682 "zon2.roo.irRadGai.dummyGlaSys.glass[1].x"; zon2_roo_irRadGai_dummyGl683 "zon2.roo.irRadGai.dummyGlaSys.glass[1].k"; zon2_roo_irRadGai_dummyGl684 "zon2.roo.irRadGai.dummyGlaSys.glass[1].tauSol"; zon2_roo_irRadGai_dummyGl685 "zon2.roo.irRadGai.dummyGlaSys.glass[1].rhoSol_a"; zon2_roo_irRadGai_dummyGl686 "zon2.roo.irRadGai.dummyGlaSys.glass[1].rhoSol_b"; zon2_roo_irRadGai_dummyGl687 "zon2.roo.irRadGai.dummyGlaSys.glass[1].tauIR"; zon2_roo_irRadGai_dummyGl688 "zon2.roo.irRadGai.dummyGlaSys.glass[1].absIR_a"; zon2_roo_irRadGai_dummyGl689 "zon2.roo.irRadGai.dummyGlaSys.glass[1].absIR_b"; zon2_roo_irRadGai_dummyGl690 "zon2.roo.irRadGai.dummyGlaSys.gas[1].x"; zon2_roo_irRadGai_dummyGl691 "zon2.roo.irRadGai.dummyGlaSys.gas[1].a_k"; zon2_roo_irRadGai_dummyGl692 "zon2.roo.irRadGai.dummyGlaSys.gas[1].b_k"; zon2_roo_irRadGai_dummyGl693 "zon2.roo.irRadGai.dummyGlaSys.gas[1].a_mu"; zon2_roo_irRadGai_dummyGl694 "zon2.roo.irRadGai.dummyGlaSys.gas[1].b_mu"; zon2_roo_irRadGai_dummyGl695 "zon2.roo.irRadGai.dummyGlaSys.gas[1].a_c"; zon2_roo_irRadGai_dummyGl696 "zon2.roo.irRadGai.dummyGlaSys.gas[1].b_c"; zon2_roo_irRadGai_dummyGl697 "zon2.roo.irRadGai.dummyGlaSys.gas[1].MM"; zon2_roo_irRadGai_dummyGl698 "zon2.roo.irRadGai.dummyGlaSys.gas[1].P0"; zon2_roo_irRadGai_dummyGl699 "zon2.roo.irRadGai.dummyGlaSys.shade.tauSol_a"; zon2_roo_irRadGai_dummyGl700 "zon2.roo.irRadGai.dummyGlaSys.shade.tauSol_b"; zon2_roo_irRadGai_dummyGl701 "zon2.roo.irRadGai.dummyGlaSys.shade.rhoSol_a"; zon2_roo_irRadGai_dummyGl702 "zon2.roo.irRadGai.dummyGlaSys.shade.rhoSol_b"; zon2_roo_irRadGai_dummyGl703 "zon2.roo.irRadGai.dummyGlaSys.shade.absIR_a"; zon2_roo_irRadGai_dummyGl704 "zon2.roo.irRadGai.dummyGlaSys.shade.absIR_b"; zon2_roo_irRadGai_dummyGl705 "zon2.roo.irRadGai.dummyGlaSys.shade.tauIR_a"; zon2_roo_irRadGai_dummyGl706 "zon2.roo.irRadGai.dummyGlaSys.shade.tauIR_b"; zon2_roo_irRadGai_dummyGl707 "zon2.roo.irRadGai.dummyGlaSys.UFra"; zon2_roo_irRadGai_dummyGl708 "zon2.roo.irRadGai.dummyGlaSys.absIRFra"; zon2_roo_irRadGai_dummyGl709 "zon2.roo.irRadGai.dummyGlaSys.absSolFra"; zon2_roo_irRadExc_datConE710 "zon2.roo.irRadExc.datConExtWin[1].ove.dep"; zon2_roo_irRadExc_datConE711 "zon2.roo.irRadExc.datConExtWin[1].sidFin.dep"; zon2_roo_irRadExc_dummyCo712 "zon2.roo.irRadExc.dummyCon.absIR_a"; zon2_roo_irRadExc_dummyCo713 "zon2.roo.irRadExc.dummyCon.absIR_b"; zon2_roo_irRadExc_dummyCo714 "zon2.roo.irRadExc.dummyCon.absSol_a"; zon2_roo_irRadExc_dummyCo715 "zon2.roo.irRadExc.dummyCon.absSol_b"; zon2_roo_irRadExc_dummyCo716 "zon2.roo.irRadExc.dummyCon.roughness_a"; zon2_roo_irRadExc_dummyGl717 "zon2.roo.irRadExc.dummyGlaSys.glass[1].x"; zon2_roo_irRadExc_dummyGl718 "zon2.roo.irRadExc.dummyGlaSys.glass[1].k"; zon2_roo_irRadExc_dummyGl719 "zon2.roo.irRadExc.dummyGlaSys.glass[1].tauSol"; zon2_roo_irRadExc_dummyGl720 "zon2.roo.irRadExc.dummyGlaSys.glass[1].rhoSol_a"; zon2_roo_irRadExc_dummyGl721 "zon2.roo.irRadExc.dummyGlaSys.glass[1].rhoSol_b"; zon2_roo_irRadExc_dummyGl722 "zon2.roo.irRadExc.dummyGlaSys.glass[1].tauIR"; zon2_roo_irRadExc_dummyGl723 "zon2.roo.irRadExc.dummyGlaSys.glass[1].absIR_a"; zon2_roo_irRadExc_dummyGl724 "zon2.roo.irRadExc.dummyGlaSys.glass[1].absIR_b"; zon2_roo_irRadExc_dummyGl725 "zon2.roo.irRadExc.dummyGlaSys.gas[1].x"; zon2_roo_irRadExc_dummyGl726 "zon2.roo.irRadExc.dummyGlaSys.gas[1].a_k"; zon2_roo_irRadExc_dummyGl727 "zon2.roo.irRadExc.dummyGlaSys.gas[1].b_k"; zon2_roo_irRadExc_dummyGl728 "zon2.roo.irRadExc.dummyGlaSys.gas[1].a_mu"; zon2_roo_irRadExc_dummyGl729 "zon2.roo.irRadExc.dummyGlaSys.gas[1].b_mu"; zon2_roo_irRadExc_dummyGl730 "zon2.roo.irRadExc.dummyGlaSys.gas[1].a_c"; zon2_roo_irRadExc_dummyGl731 "zon2.roo.irRadExc.dummyGlaSys.gas[1].b_c"; zon2_roo_irRadExc_dummyGl732 "zon2.roo.irRadExc.dummyGlaSys.gas[1].MM"; zon2_roo_irRadExc_dummyGl733 "zon2.roo.irRadExc.dummyGlaSys.gas[1].P0"; zon2_roo_irRadExc_dummyGl734 "zon2.roo.irRadExc.dummyGlaSys.shade.tauSol_a"; zon2_roo_irRadExc_dummyGl735 "zon2.roo.irRadExc.dummyGlaSys.shade.tauSol_b"; zon2_roo_irRadExc_dummyGl736 "zon2.roo.irRadExc.dummyGlaSys.shade.rhoSol_a"; zon2_roo_irRadExc_dummyGl737 "zon2.roo.irRadExc.dummyGlaSys.shade.rhoSol_b"; zon2_roo_irRadExc_dummyGl738 "zon2.roo.irRadExc.dummyGlaSys.shade.absIR_a"; zon2_roo_irRadExc_dummyGl739 "zon2.roo.irRadExc.dummyGlaSys.shade.absIR_b"; zon2_roo_irRadExc_dummyGl740 "zon2.roo.irRadExc.dummyGlaSys.shade.tauIR_a"; zon2_roo_irRadExc_dummyGl741 "zon2.roo.irRadExc.dummyGlaSys.shade.tauIR_b"; zon2_roo_irRadExc_dummyGl742 "zon2.roo.irRadExc.dummyGlaSys.UFra"; zon2_roo_irRadExc_dummyGl743 "zon2.roo.irRadExc.dummyGlaSys.absIRFra"; zon2_roo_irRadExc_dummyGl744 "zon2.roo.irRadExc.dummyGlaSys.absSolFra"; zon2_roo_irRadExc_T0 "zon2.roo.irRadExc.T0"; zon2_roo_radTem_datConExt746 "zon2.roo.radTem.datConExtWin[1].ove.dep"; zon2_roo_radTem_datConExt747 "zon2.roo.radTem.datConExtWin[1].sidFin.dep"; zon2_roo_radTem_dummyCon_748 "zon2.roo.radTem.dummyCon.absIR_a"; zon2_roo_radTem_dummyCon_749 "zon2.roo.radTem.dummyCon.absIR_b"; zon2_roo_radTem_dummyCon_750 "zon2.roo.radTem.dummyCon.absSol_a"; zon2_roo_radTem_dummyCon_751 "zon2.roo.radTem.dummyCon.absSol_b"; zon2_roo_radTem_dummyCon_752 "zon2.roo.radTem.dummyCon.roughness_a"; zon2_roo_radTem_dummyGlaS753 "zon2.roo.radTem.dummyGlaSys.glass[1].x"; zon2_roo_radTem_dummyGlaS754 "zon2.roo.radTem.dummyGlaSys.glass[1].k"; zon2_roo_radTem_dummyGlaS755 "zon2.roo.radTem.dummyGlaSys.glass[1].tauSol"; zon2_roo_radTem_dummyGlaS756 "zon2.roo.radTem.dummyGlaSys.glass[1].rhoSol_a"; zon2_roo_radTem_dummyGlaS757 "zon2.roo.radTem.dummyGlaSys.glass[1].rhoSol_b"; zon2_roo_radTem_dummyGlaS758 "zon2.roo.radTem.dummyGlaSys.glass[1].tauIR"; zon2_roo_radTem_dummyGlaS759 "zon2.roo.radTem.dummyGlaSys.glass[1].absIR_a"; zon2_roo_radTem_dummyGlaS760 "zon2.roo.radTem.dummyGlaSys.glass[1].absIR_b"; zon2_roo_radTem_dummyGlaS761 "zon2.roo.radTem.dummyGlaSys.gas[1].x"; zon2_roo_radTem_dummyGlaS762 "zon2.roo.radTem.dummyGlaSys.gas[1].a_k"; zon2_roo_radTem_dummyGlaS763 "zon2.roo.radTem.dummyGlaSys.gas[1].b_k"; zon2_roo_radTem_dummyGlaS764 "zon2.roo.radTem.dummyGlaSys.gas[1].a_mu"; zon2_roo_radTem_dummyGlaS765 "zon2.roo.radTem.dummyGlaSys.gas[1].b_mu"; zon2_roo_radTem_dummyGlaS766 "zon2.roo.radTem.dummyGlaSys.gas[1].a_c"; zon2_roo_radTem_dummyGlaS767 "zon2.roo.radTem.dummyGlaSys.gas[1].b_c"; zon2_roo_radTem_dummyGlaS768 "zon2.roo.radTem.dummyGlaSys.gas[1].MM"; zon2_roo_radTem_dummyGlaS769 "zon2.roo.radTem.dummyGlaSys.gas[1].P0"; zon2_roo_radTem_dummyGlaS770 "zon2.roo.radTem.dummyGlaSys.shade.tauSol_a"; zon2_roo_radTem_dummyGlaS771 "zon2.roo.radTem.dummyGlaSys.shade.tauSol_b"; zon2_roo_radTem_dummyGlaS772 "zon2.roo.radTem.dummyGlaSys.shade.rhoSol_a"; zon2_roo_radTem_dummyGlaS773 "zon2.roo.radTem.dummyGlaSys.shade.rhoSol_b"; zon2_roo_radTem_dummyGlaS774 "zon2.roo.radTem.dummyGlaSys.shade.absIR_a"; zon2_roo_radTem_dummyGlaS775 "zon2.roo.radTem.dummyGlaSys.shade.absIR_b"; zon2_roo_radTem_dummyGlaS776 "zon2.roo.radTem.dummyGlaSys.shade.tauIR_a"; zon2_roo_radTem_dummyGlaS777 "zon2.roo.radTem.dummyGlaSys.shade.tauIR_b"; zon2_roo_radTem_dummyGlaS778 "zon2.roo.radTem.dummyGlaSys.UFra"; zon2_roo_radTem_dummyGlaS779 "zon2.roo.radTem.dummyGlaSys.absIRFra"; zon2_roo_radTem_dummyGlaS780 "zon2.roo.radTem.dummyGlaSys.absSolFra"; zon2_roo_add_k1 "zon2.roo.add.k1"; zon2_roo_add_k2 "zon2.roo.add.k2"; zon2_roo_sumJFroWin_1__k "zon2.roo.sumJFroWin[1].k"; zon2_roo_p_start "zon2.roo.p_start"; zon2_roo_T_start "zon2.roo.T_start"; zon2_roo_X_start "zon2.roo.X_start"; zon2_qConGai_flow_k "zon2.qConGai_flow.k"; zon2_qRadGai_flow_k "zon2.qRadGai_flow.k"; zon2_qLatGai_flow_k "zon2.qLatGai_flow.k"; zon2_TSoi_1__T "zon2.TSoi[1].T"; zon2_sinInf_m_flow "zon2.sinInf.m_flow"; zon2_sinInf_x_pTphi_p "zon2.sinInf.x_pTphi.p"; zon2_InfiltrationRate_k "zon2.InfiltrationRate.k"; zon2_souInf_m_flow "zon2.souInf.m_flow"; zon2_souInf_x_pTphi_p "zon2.souInf.x_pTphi.p"; zon2_intLoad_table "zon2.intLoad.table"; zon2_intLoad_verboseRead "zon2.intLoad.verboseRead"; zon2_intLoad_columns "zon2.intLoad.columns"; zon2_intLoad_offset "zon2.intLoad.offset"; zon2_intLoad_startTime "zon2.intLoad.startTime"; zon2_intLoad_timeEvents "zon2.intLoad.timeEvents"; zon1_roo_conExtWin_1__win802 "zon1.roo.conExtWin[1].win.glaUns.glass[1].T0"; zon1_roo_conExtWin_1__win803 "zon1.roo.conExtWin[1].win.glaUns.glass[2].T0"; zon1_roo_conExtWin_1__win804 "zon1.roo.conExtWin[1].win.glaUns.gas[1].T0"; zon2_roo_conExtWin_1__win805 "zon2.roo.conExtWin[1].win.glaUns.glass[1].T0"; zon2_roo_conExtWin_1__win806 "zon2.roo.conExtWin[1].win.glaUns.glass[2].T0"; zon2_roo_conExtWin_1__win807 "zon2.roo.conExtWin[1].win.glaUns.gas[1].T0"
      mask Display: image(imread('Dymola.bmp'))
  compmodel : Subsystem
      settings: OpenFcn=compileModelica('twozonevav/behavior/dymola');
      mask Display: disp('Compile Modelica model');
  editmodel : Subsystem
      settings: OpenFcn=editModelica('twozonevav/behavior/dymola');
      mask Display: disp('Edit Modelica model');
  TRooAir1 : Outport
  TDis1 : Outport  Port=2
  V1_flow : Outport  Port=3
  TDis2 : Outport  Port=4
  TRooAir2 : Outport  Port=5
  V2_flow : Outport  Port=6
  weaBus_HDifHor : Outport  Port=7
  weaBus_HDirNor : Outport  Port=8
  weaBus_HGloHor : Outport  Port=9
  weaBus_HHorIR : Outport  Port=10
  weaBus_TBlaSky : Outport  Port=11
  weaBus_TDewPoi : Outport  Port=12
  weaBus_TDryBul : Outport  Port=13
  weaBus_ceiHei : Outport  Port=14
  weaBus_cloTim : Outport  Port=15
  weaBus_lat : Outport  Port=16
  weaBus_lon : Outport  Port=17
  weaBus_nOpa : Outport  Port=18
  weaBus_nTot : Outport  Port=19
  weaBus_pAtm : Outport  Port=20
  weaBus_relHum : Outport  Port=21
  weaBus_solAlt : Outport  Port=22
  weaBus_solDec : Outport  Port=23
  weaBus_solHouAng : Outport  Port=24
  weaBus_solTim : Outport  Port=25
  weaBus_solZen : Outport  Port=26
  weaBus_winDir : Outport  Port=27
  weaBus_winSpe : Outport  Port=28
  wires:
  Sfunc/1 -> Demux/1
  Demux/1 -> TRooAir1/1
  Demux/2 -> TDis1/1
  Demux/3 -> V1_flow/1
  Demux/4 -> TDis2/1
  Demux/5 -> TRooAir2/1
  Demux/6 -> V2_flow/1
  Demux/7 -> weaBus_HDifHor/1
  Demux/8 -> weaBus_HDirNor/1
  Demux/9 -> weaBus_HGloHor/1
  Demux/10 -> weaBus_HHorIR/1
  Demux/11 -> weaBus_TBlaSky/1
  Demux/12 -> weaBus_TDewPoi/1
  Demux/13 -> weaBus_TDryBul/1
  Demux/14 -> weaBus_ceiHei/1
  Demux/15 -> weaBus_cloTim/1
  Demux/16 -> weaBus_lat/1
  Demux/17 -> weaBus_lon/1
  Demux/18 -> weaBus_nOpa/1
  Demux/19 -> weaBus_nTot/1
  Demux/20 -> weaBus_pAtm/1
  Demux/21 -> weaBus_relHum/1
  Demux/22 -> weaBus_solAlt/1
  Demux/23 -> weaBus_solDec/1
  Demux/24 -> weaBus_solHouAng/1
  Demux/25 -> weaBus_solTim/1
  Demux/26 -> weaBus_solZen/1
  Demux/27 -> weaBus_winDir/1
  Demux/28 -> weaBus_winSpe/1
  Mux/1 -> Sfunc/1
  yVAV1/1 -> Mux/1
  yVAV2/1 -> Mux/2
